simulink model "OMAP_ver_MIL10"  (R2018b)
settings: Solver=FixedStepDiscrete  StartTime=0.0  StopTime=10.0  FixedStep=0.01  RelTol=1e-3
undefined symbols (not defined in the file or in its folder): OMAP_Switch_EMS, OMAP_Switch_EPS, OMAP_Switch_ESC, OMAP_Switch_IC, OMAP_Switch_OTHER, TH_HMIClb_tiDgrdIconWarnHiDurT_C, TH_HMIClb_tiDgrdIconWarnLoDurT_C, TH_HMIClb_tiDgrdVocWarnDurT_C, TH_HMIClb_tiHndOffTxtWarnT_C, TH_HMIClb_tiHndOffVocWarnT_C, TH_HMIClb_tiSWALimFlgDetT_C, TH_HMIClb_tiTxtLimT_C
libraries: simulink x118
(part 2 of 9)

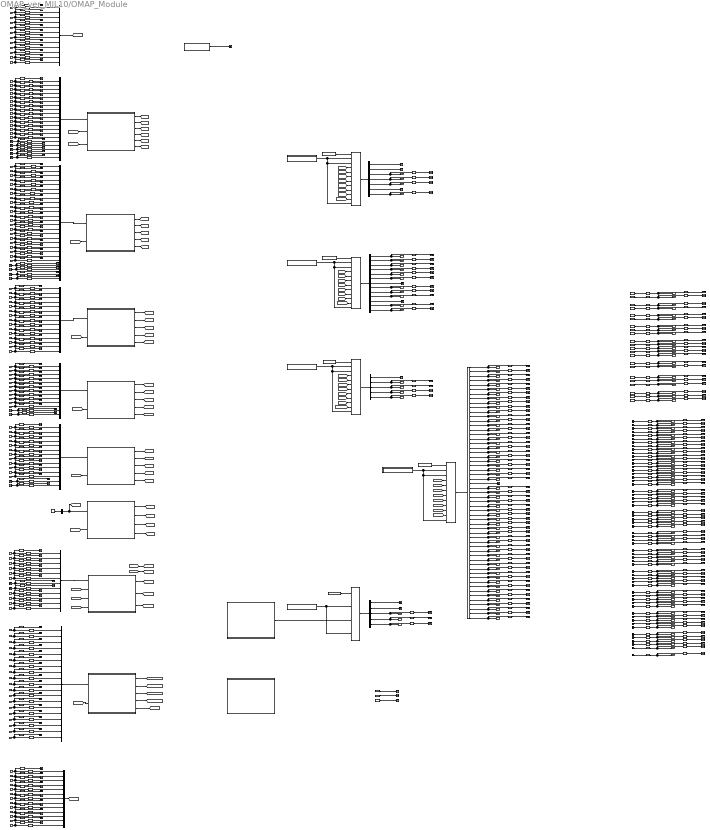
== system OMAP_ver_MIL10/OMAP_Module ==
  note: 仲裁#19——EW单功能调试模式
      | EMS、ESC、EPS、IC：只体现本功能的信号、且其他信号内容强制为“不动作”
  note: 仲裁#12——ACC单功能调试模式
      | EMS、ESC、EPS、IC：只体现本功能的信号、且其他信号内容强制为“不动作”
  note: 仲裁#17——ESA单功能调试模式
      | EMS、ESC、EPS、IC：只体现本功能的信号、且其他信号内容强制为“不动作”
  note: 仲裁#13——AEB单功能调试模式
      | EMS、ESC、EPS、IC：只体现本功能的信号、且其他信号内容强制为“不动作”
  note: 上面这是版本号
      | 蓝色的子系统是输入，橙色是仲裁输出，
      | 翠绿色的模块是标定量
  note: 仲裁#18——ICA单功能调试模式
      | EMS、ESC：只体现ACC的信号、且其他信号内容强制为“不动作”
      | EPS：只体现本功能的信号、且其他信号内容强制为“不动作”
      | IC：只体现本功能及ACC综合后的的信号、且其他信号内容强制为“不动作”
  note: 仲裁#16——ELK单功能调试模式
      | EMS、ESC、EPS、IC：只体现本功能的信号、且其他信号内容强制为“不动作”
  note: 仲裁#15——LKA单功能调试模式
      | EMS、ESC、EPS、IC：只体现本功能的信号、且其他信号内容强制为“不动作”
  note: 仲裁#14——JA单功能调试模式——
      | EMS、ESC、EPS、IC：只体现本功能的信号、且其他信号内容强制为“不动作”
  FDMMve_d_JaFcnConf : Inport  OutDataTypeStr=uint16
  FDMMve_d_AebFcnConf : Inport  Port=2  OutDataTypeStr=uint16
  FDMMve_d_EsaFcnConf : Inport  Port=3  OutDataTypeStr=uint16
  FDMMve_d_ElkFcnConf : Inport  Port=4  OutDataTypeStr=uint16
  FDMMve_d_LkaFcnConf : Inport  Port=5  OutDataTypeStr=uint16
  FDMMve_d_IcaFcnConf : Inport  Port=6  OutDataTypeStr=uint16
  FDMMve_d_AccFcnConf : Inport  Port=7  OutDataTypeStr=uint16
  FDMMve_d_LfFcnConf : Inport  Port=8  OutDataTypeStr=uint16
  FDMMve_d_AlcFcnConf : Inport  Port=9  OutDataTypeStr=uint16
  FDMMve_d_EwFcnConf : Inport  Port=10  OutDataTypeStr=uint16
  FDMMve_g_Adas2Fapa : Inport  Port=11  OutDataTypeStr=uint32
  FDMMve_d_SignalTStamp : Inport  Port=12  OutDataTypeStr=uint16
  ACCSve_d_ACC_State : Inport  Port=13  OutDataTypeStr=uint16
  ACCSve_g_ACC_TqReq : Inport  Port=14  OutDataTypeStr=single
  ACCSve_d_ACC_TqFlag : Inport  Port=15  OutDataTypeStr=uint16
  ACCSve_g_ACC_DecReq : Inport  Port=16  OutDataTypeStr=single
  ACCSve_d_ACC_DecFlag : Inport  Port=17  OutDataTypeStr=uint16
  ACCSve_d_CIPV_ID : Inport  Port=18  OutDataTypeStr=uint16
  ACCSve_d_ACCActive_Signal : Inport  Port=19  OutDataTypeStr=uint16
  ACCSve_d_ACC_go_request : Inport  Port=20  OutDataTypeStr=uint16
  ACCSve_d_VelocitySet : Inport  Port=21  OutDataTypeStr=uint16
  ACCSve_d_HeadWaySet : Inport  Port=22  OutDataTypeStr=uint16
  ACCSve_d_SignalTStamp : Inport  Port=23  OutDataTypeStr=uint16
  ACCSve_d_ACC_ICA_Flag : Inport  Port=24  OutDataTypeStr=uint16
  ACCSve_d_ACC_ESCDriveOff : Inport  Port=25  OutDataTypeStr=uint16
  ACCSve_d_ACC_ESCHoldReq : Inport  Port=26  OutDataTypeStr=uint16
  ACCSve_d_ACC_EPBReq : Inport  Port=27  OutDataTypeStr=uint16
  AEBSve_d_Prefill_request : Inport  Port=28  OutDataTypeStr=uint16
  AEBSve_d_functionFARCState : Inport  Port=29  OutDataTypeStr=uint16
  AEBSve_g_DecSetpoint : Inport  Port=30  OutDataTypeStr=single
  AEBSve_d_MDDdecRequest : Inport  Port=31  OutDataTypeStr=uint16
  AEBSve_d_MDDdecType : Inport  Port=32  OutDataTypeStr=uint16
  AEBSve_d_ESCDriveOff : Inport  Port=33  OutDataTypeStr=uint16
  AEBSve_d_ESCHoldReq : Inport  Port=34  OutDataTypeStr=uint16
  AEBSve_d_HapticAlarm : Inport  Port=35  OutDataTypeStr=uint16
  AEBSve_d_Braking_progress : Inport  Port=36  OutDataTypeStr=uint16
  AEBSve_d_AEBStatus : Inport  Port=37  OutDataTypeStr=uint16
  AEBSve_d_FCWStatus : Inport  Port=38  OutDataTypeStr=uint16
  AEBSve_d_AEBSwitchStatus : Inport  Port=39  OutDataTypeStr=uint16
  AEBSve_d_AEBFaultStatus : Inport  Port=40  OutDataTypeStr=uint16
  AEBSve_d_AEBAlertReq : Inport  Port=41  OutDataTypeStr=uint16
  AEBSve_d_AEBTips : Inport  Port=42  OutDataTypeStr=uint16
  AEBSve_d_SignalTStamp : Inport  Port=43  OutDataTypeStr=uint16
  AEBSve_d_JABS_AlertSign : Inport  Port=44  OutDataTypeStr=uint16
  AEBSve_d_JABS_SwitchStatus : Inport  Port=45  OutDataTypeStr=uint16
  AEBSve_d_JABS_FltStatus : Inport  Port=46  OutDataTypeStr=uint16
  AEBSve_d_JABS_AlertReq : Inport  Port=47  OutDataTypeStr=uint16
  AEBSve_d_JABS_HapticAlarm : Inport  Port=48  OutDataTypeStr=uint16
  AEBSve_d_JABS_Tips : Inport  Port=49  OutDataTypeStr=uint16
  JABSve_d_DbPrefillReq : Inport  Port=50  OutDataTypeStr=uint16
  JABSve_d_DbFunFARCSta : Inport  Port=51  OutDataTypeStr=uint16
  JABSve_g_DbDecSetpoint : Inport  Port=52  OutDataTypeStr=single
  JABSve_d_DbMDDdecRequest : Inport  Port=53  OutDataTypeStr=uint16
  JABSve_d_DbMDDdecType : Inport  Port=54  OutDataTypeStr=uint16
  JABSve_d_DbHapticAlarm : Inport  Port=55  OutDataTypeStr=uint16
  JABSve_d_DbBraking_progress : Inport  Port=56  OutDataTypeStr=uint16
  JABSve_d_DbSignalTStamp : Inport  Port=57  OutDataTypeStr=uint16
  JABSve_d_DbJACWStatus : Inport  Port=58  OutDataTypeStr=uint16
  JABSve_d_DbSwitchStatus : Inport  Port=59  OutDataTypeStr=uint16
  JABSve_d_DbFltStatus : Inport  Port=60  OutDataTypeStr=uint16
  JABSve_d_DbAlertReq : Inport  Port=61  OutDataTypeStr=uint16
  JABSve_d_DbTips : Inport  Port=62  OutDataTypeStr=uint16
  JABSve_d_DbESCDriveOff : Inport  Port=63  OutDataTypeStr=uint16
  JABSve_d_DbESCHoldReq : Inport  Port=64  OutDataTypeStr=uint16
  LKASve_y_Vehicle_Lane_Display : Inport  Port=65  OutDataTypeStr=uint8
  LKASve_y_LDW_Status_Display : Inport  Port=66  OutDataTypeStr=uint8
  LKASve_y_LKA_Status_Display : Inport  Port=67  OutDataTypeStr=uint8
  LKASve_y_LDW_Flag : Inport  Port=68  OutDataTypeStr=uint8
  LKASve_y_Hands_Off_Warning : Inport  Port=69  OutDataTypeStr=uint8
  LKASve_y_LKA_Action_Indication : Inport  Port=70  OutDataTypeStr=uint8
  LKASve_y_HMI_Popup_Status : Inport  Port=71  OutDataTypeStr=uint8
  LKASve_y_EPS_State_Control : Inport  Port=72  OutDataTypeStr=uint8
  LKASve_g_LKA_SWA_Control : Inport  Port=73  OutDataTypeStr=single
  LKASve_g_EPS_Factor_Control : Inport  Port=74  OutDataTypeStr=single
  LKASve_y_EPS_LKA_Control : Inport  Port=75  OutDataTypeStr=uint8
  ELKSve_y_state_ELK_function : Inport  Port=76  OutDataTypeStr=uint8
  ELKSve_y_ELK_HapticAlarmReq : Inport  Port=77  OutDataTypeStr=uint8
  ELKSve_y_Hands_Off_Warning : Inport  Port=78  OutDataTypeStr=uint8
  ELKSve_y_ELK_Action_Indication : Inport  Port=79  OutDataTypeStr=uint8
  ELKSve_y_HMI_Popup_Status : Inport  Port=80  OutDataTypeStr=uint8
  ELKSve_y_EPS_State_Control : Inport  Port=81  OutDataTypeStr=uint8
  ELKSve_g_ELK_SWA_Control : Inport  Port=82  OutDataTypeStr=single
  ELKSve_g_EPS_Factor_Control : Inport  Port=83  OutDataTypeStr=single
  ELKSve_y_EPS_ELK_Control : Inport  Port=84  OutDataTypeStr=uint8
  ELKSve_y_ELK_VehicleLaneDisp : Inport  Port=85  OutDataTypeStr=uint8
  ELKSve_y_ELK_ELKSts : Inport  Port=86  OutDataTypeStr=uint8
  ELKSve_y_SignalTStamp : Inport  Port=87  OutDataTypeStr=uint8
  ICABva_d_PathQI : Inport  Port=88  OutDataTypeStr=uint16
  ICABve_d_SignalTStamp : Inport  Port=89  OutDataTypeStr=uint16
  ICABva_d_ICAB2HMI : Inport  Port=90  OutDataTypeStr=uint16
  ICABve_g_SteerAngleCmd : Inport  Port=91  OutDataTypeStr=single
  ICABve_d_ICAMode : Inport  Port=92  OutDataTypeStr=uint16
  ICABve_d_ICAState : Inport  Port=93  OutDataTypeStr=uint16
  ICADva_d_DecionState : Inport  Port=94  OutDataTypeStr=uint16
  ICADva_d_DecionCMD : Inport  Port=95  OutDataTypeStr=uint16
  ICADva_d_LCRecommend : Inport  Port=96  OutDataTypeStr=uint16
  ICADve_d_SignalTStamp : Inport  Port=97  OutDataTypeStr=uint16
  EWWWve_y_LCW_M_SystemWorkingSt : Inport  Port=98  OutDataTypeStr=uint8
  EWWWve_y_RCTA_M_SystemWorkingSt : Inport  Port=99  OutDataTypeStr=uint8
  EWWWve_y_DOW_M_SystemWorkingSt : Inport  Port=100  OutDataTypeStr=uint8
  EWWWve_y_BSD_M_ErrorSt : Inport  Port=101  OutDataTypeStr=uint8
  EWWWve_y_BSD_M_LCAWarning : Inport  Port=102  OutDataTypeStr=uint8
  EWWWve_y_BSD_M_DoorOpenWarning : Inport  Port=103  OutDataTypeStr=uint8
  EWWWve_y_BSD_M_RCTAWarning : Inport  Port=104  OutDataTypeStr=uint8
  EWWWve_y_BSD_S_LCAWarning : Inport  Port=105  OutDataTypeStr=uint8
  EWWWve_y_BSD_S_DoorOpenWarning : Inport  Port=106  OutDataTypeStr=uint8
  EWWWve_y_BSD_S_RCTAWarning : Inport  Port=107  OutDataTypeStr=uint8
  EWWWve_y_SRR_LF_FCTAWorkingSt : Inport  Port=108  OutDataTypeStr=uint8
  EWWWve_y_SRR_LF_ErrorSt : Inport  Port=109  OutDataTypeStr=uint8
  EWWWve_y_SRR_LF_FCTAWarning : Inport  Port=110  OutDataTypeStr=uint8
  EWWWve_y_SRR_RF_FCTAWarning : Inport  Port=111  OutDataTypeStr=uint8
  EWWWve_y_SRR_SystemState : Inport  Port=112  OutDataTypeStr=uint8
  EWWWve_y_BSD_S_SystemStateInfo : Inport  Port=113  OutDataTypeStr=uint8
  EWWWve_y_BSD_SystemStateInfo : Inport  Port=114  OutDataTypeStr=uint8
  EWWWve_y_SRR_LF_SystemStateInfo : Inport  Port=115  OutDataTypeStr=uint8
  EWWWve_y_SRR_RF_SystemStateInfo : Inport  Port=116  OutDataTypeStr=uint8
  IMAPve_d_EPS_LKA_State : Inport  Port=117  OutDataTypeStr=uint16
  IMAPve_g_ESC_LonAcc : Inport  Port=118  OutDataTypeStr=single
  IMAPva_d_obj_id : Inport  Port=119  OutDataTypeStr=uint16
  IMAPva_g_obj_pos_x : Inport  Port=120  OutDataTypeStr=single
  IMAPve_d_ESC_Veh_Standstill : Inport  Port=121  OutDataTypeStr=uint16
  IMAPve_g_L0_C0 : Inport  Port=122  OutDataTypeStr=single
  IMAPve_g_L0_C1 : Inport  Port=123  OutDataTypeStr=single
  IMAPve_g_L0_C2 : Inport  Port=124  OutDataTypeStr=single
  IMAPve_g_L0_C3 : Inport  Port=125  OutDataTypeStr=single
  IMAPve_g_R0_C0 : Inport  Port=126  OutDataTypeStr=single
  IMAPve_g_R0_C1 : Inport  Port=127  OutDataTypeStr=single
  IMAPve_g_R0_C2 : Inport  Port=128  OutDataTypeStr=single
  IMAPve_g_R0_C3 : Inport  Port=129  OutDataTypeStr=single
  ACCS_Direct : Subsystem
  AEBS_Direct : Subsystem
  Bus Creator : BusCreator  Inputs=1
  Bus Selector : BusSelector  OutputSignals=OMAPve_y_ACC_Engine_Start_Request_1,OMAPve_g_PotACCTqReq_1,OMAPve_g_ACCTqReq_1,OMAPve_y_Powertrain_torquewheel_request_1,OMAPve_g_TminUp_or_downGear_1,OMAPve_y_stAcvTqWhlPTPotReq_1,OMAPve_y_Function_Acc_status_1
  Bus Selector1 : BusSelector  OutputSignals=OMAPve_g_Deceleration_setpoint_device_1,OMAPve_y_MDD_Decelerationcontrol_request_1,OMAPve_y_Prefill_request_1,OMAPve_y_ADAS_ESCDriveOff,OMAPve_y_ADAS_ESCHoldReq,OMAPve_y_MDD_deceleration_type_1,OMAPve_y_State_of_the_functionFARC_det_1,OMAPve_y_AEB_Status_1,OMAPve_y_Decel_Request_1,OMAPve_y_AEB_Braking_progress_1,OMAPve_y_FCW_Status_1,OMAPve_y_Haptic_Alarm_1,OMAPve_y_ADAS_ACCRequestEPB
  Bus Selector2 : BusSelector  OutputSignals=OMAPve_y_Power_steering_power_cut3F2_2,OMAPve_y_General_state_of_LKA_function3F2_2,OMAPve_g_Coefficient_toregulate_EPS_2,OMAPve_g_Column_angle_setpoint3F2_2,OMAPve_y_Permit_to_know_if_LKA_or_LPA3F2_2
  Bus Selector3 : BusSelector  OutputSignals=OMAPve_y_TSR_Vision_Only_Sign_Type_2,OMAPve_y_ISA_Popup_text_2,OMAPve_y_ISA_Sign_Type_2,OMAPve_y_ISA_Status_2,OMAPve_y_ISA_Value_2,OMAPve_y_ACC_DesiredHeadway_Display_2,OMAPve_y_ACC_DesiredHeadway_Icon_Basic_2,OMAPve_y_ACC_Desired_Set_Speed_2,OMAPve_y_ACC_Set_Speed_Display_2,OMAPve_y_ACC_Vehicle_Icon_Display_2,OMAPve_y_RVVACC_Vehiclespeed_request_type_2,OMAPve_y_ACC_Pop_Up_Message_2,OMAPve_y_AEB_Alert_Req_2,OMAPve_y_AEB_Fault_Status_2,OMAPve_y_AEB_Switch_Status_2,OMAPve_y_AEB_tips_2,OMAPve_y_ACC_HMI_TgtDisp_Flag_2,OMAPve_y_TARGET_POSITION_2,OMAPve_y_Hands_off_warning_2,OMAPve_y_HMI_Popup_Status_2,OMAPve_y_Vehicle_Lane_Display_2,OMAPve_y_LDW_Flag_2,OMAPve_y_LDW_Status_Display_2,OMAPve_y_LKA_Mode_from_Camera_2,OMAPve_y_LKA_Status_Display_2,OMAPve_y_LKA_Switch_State_2,OMAPve_y_LKA_action_indication_2,OMAPve_y_ADAS_ELKSts_2,OMAPve_y_ICA_HMI_Txt_Disp_2,OMAPve_y_TJA_status_icon_2,OMAPve_y_ADAS_SRR_SystemState,OMAPve_y_ADAS_LeftLEDWarningSt,OMAPve_y_ADAS_RighrLEDWarningSt,OMAPve_y_ADAS_BSD_SystemStInfo,OMAPve_y_ADAS_BSD_LCWWorkingSt,OMAPve_y_ADAS_BSD_ErrorSt,OMAPve_y_ADAS_BSD_LCAWarning,OMAPve_y_ADAS_BSD_DoorOpenWrn,OMAPve_y_ADAS_BSD_RCTAWarning,OMAPve_y_ADAS_BSD_DOWWorkingSt,OMAPve_y_ADAS_BSD_RCTAWorkingSt,OMAPve_y_ADAS_BSD_S_SystStInfo,OMAPve_y_ADAS_BSD_S_LCWWorkSt,OMAPve_y_ADAS_BSD_S_ErrorSt,OMAPve_y_ADAS_BSD_S_LCAWarning,OMAPve_y_ADAS_BSD_S_DoorOpenWrn,OMAPve_y_ADAS_BSD_S_RCTAWarning,OMAPve_y_ADAS_BSD_S_DOWWorkSt,OMAPve_y_ADAS_BSD_S_RCTAWorkSt,OMAPve_y_ADAS_SRR_LF_SystStInfo,OMAPve_y_ADAS_SRR_LF_SystWorkSt,OMAPve_y_ADAS_SRR-LF_ErrorSt,OMAPve_y_ADAS_SRR_LF_FCTAWrn,OMAPve_y_ADAS_SRR_RF_SystStInfo,OMAPve_y_ADAS_SRR_RF_SystWorkSt,OMAPve_y_ADAS_SRR-RF_ErrorSt,OMAPve_y_ADAS_SRR_RF_FCTAWrn
  Bus Selector4 : BusSelector  OutputSignals=OMAPve_y_ABS_ESP_power_cut_request2_2,OMAPve_y_ASR_connection_dis_demand2_2,OMAPve_y_TYPE_RAPPORT_2,OMAPve_y_ECU_operating_phase_2,OMAPve_y_Radar_State_2
  Bus_ACCS : BusCreator  Inputs=20
  Bus_AEBS : BusCreator  Inputs=26
  Bus_ELKS : BusCreator  Inputs=14
  Bus_EW : BusCreator  Inputs=19
  Bus_FDMM : BusCreator  Inputs=12
  Bus_ICA : BusCreator  Inputs=12
  Bus_IMAP : BusCreator  Inputs=13
  Bus_JABS : BusCreator  Inputs=15
  Bus_LKAS : BusCreator  Inputs=13
  CHecksum_Rollingcounter : Subsystem
  Constant : Constant  Value=OMAP_Switch_EMS  OutDataTypeStr=uint8
  Constant1 : Constant  Value=OMAP_Switch_ESC  OutDataTypeStr=uint8
  Constant2 : Constant  Value=OMAP_Switch_EPS  OutDataTypeStr=uint8
  Constant3 : Constant  Value=OMAP_Switch_IC  OutDataTypeStr=uint8
  Constant4 : Constant  Value=OMAP_Switch_OTHER  OutDataTypeStr=uint8
  Constant5 : Constant  OutDataTypeStr=uint8
  Constant6 : Constant  Value=920  OutDataTypeStr=uint16
  Data Type Conversion{,1..10,13..21,23..31,55,57..58,60,62..63,78..86,89..91,93,95..98,100,149..160,162..165,167..177,180} (81 alike) : DataTypeConversion  OutDataTypeStr=uint16
  Data Type Conversion{54,56,88,92,94,99,101..110,144..145,161,166,179,182} (22 alike) : DataTypeConversion  OutDataTypeStr=single
  Data Type Conversion{11..12,87,111..143,146..148,178} (40 alike) : DataTypeConversion  OutDataTypeStr=uint8
  Data Type Conversion22 : DataTypeConversion  OutDataTypeStr=uint32
  Default_EMS : Subsystem
  Default_EPS : Subsystem
  Default_ESC : Subsystem
  Default_IC : Subsystem
  Default_OTHER : Subsystem
  ELKS_Direct : Subsystem
  ESAS_Direct : Subsystem
  EW_ISA_TSR_Direct : Subsystem
  Ground{,1..14} (15 alike) : Ground
  ICA_Direct_G59 : Subsystem
  Index Vector{,1..3} (4 alike) : MultiPortSwitch  DataPortOrder=Zero-based contiguous  Inputs=11  zeroidx=on
  Index Vector4 : MultiPortSwitch  DataPortOrder=Zero-based contiguous  zeroidx=on
  JABS_Direct : Subsystem
  LKAS_Direct : Subsystem
  OMAPve_g_ADAS_ESATorqueReq1 : Constant  Value=0  OutDataTypeStr=single
  OMAPve_g_ADAS_L0_C0_COEF_2 : Ground
  OMAPve_g_ADAS_L0_C1_COEF_2 : Ground
  OMAPve_g_ADAS_L0_C2_COEF_2 : Ground
  OMAPve_g_ADAS_L0_C3_COEF_2 : Ground
  OMAPve_g_ADAS_OBJ01_LatDis_2 : Ground
  OMAPve_g_ADAS_OBJ01_LgtDis_2 : Ground
  OMAPve_g_ADAS_OBJ02_LatDis_2 : Ground
  OMAPve_g_ADAS_OBJ02_LgtDis_2 : Ground
  OMAPve_g_ADAS_OBJ03_LatDis_2 : Ground
  OMAPve_g_ADAS_OBJ03_LgtDis_2 : Ground
  OMAPve_g_ADAS_OBJ04_LatDis_2 : Ground
  OMAPve_g_ADAS_OBJ04_LgtDis_2 : Ground
  OMAPve_g_ADAS_OBJ05_LatDis_2 : Ground
  OMAPve_g_ADAS_OBJ05_LgtDis_2 : Ground
  OMAPve_g_ADAS_OBJ06_LatDis_2 : Ground
  OMAPve_g_ADAS_OBJ06_LgtDis_2 : Ground
  OMAPve_g_ADAS_R0_C0_COEF_2 : Ground
  OMAPve_g_ADAS_R0_C1_COEF_2 : Ground
  OMAPve_g_ADAS_R0_C2_COEF_2 : Ground
  OMAPve_g_ADAS_R0_C3_COEF_2 : Ground
  OMAPve_y_ADAS_ACCLateralDist1 : Constant  Value=0  OutDataTypeStr=int8
  OMAPve_y_ADAS_ACCLongiDist1 : Constant  Value=0  OutDataTypeStr=uint8
  OMAPve_y_ADAS_BackObjectLeft_2 : Ground
  OMAPve_y_ADAS_BackObjectRight_2 : Ground
  OMAPve_y_ADAS_ESAFaultSt1 : Constant  Value=0  OutDataTypeStr=uint8
  OMAPve_y_ADAS_ESARequest1 : Constant  Value=0  OutDataTypeStr=uint8
  OMAPve_y_ADAS_ESAState1 : Constant  Value=0  OutDataTypeStr=uint8
  OMAPve_y_ADAS_EngStartReqForSTT1 : Constant  Value=0  OutDataTypeStr=uint8
  OMAPve_y_ADAS_EngStopPmtForSTT1 : Constant  Value=0  OutDataTypeStr=uint8
  OMAPve_y_ADAS_FrontObj01Class_2 : Ground
  OMAPve_y_ADAS_FrontObj02Class_2 : Ground
  OMAPve_y_ADAS_FrontObj03Class_2 : Ground
  OMAPve_y_ADAS_FrontObj04Class_2 : Ground
  OMAPve_y_ADAS_FrontObj05Class_2 : Ground
  OMAPve_y_ADAS_FrontObj06Class_2 : Ground
  OMAPve_y_ADAS_FrontObject01Zone_2 : Ground
  OMAPve_y_ADAS_FrontObject02Zone_2 : Ground
  OMAPve_y_ADAS_FrontObject03Zone_2 : Ground
  OMAPve_y_ADAS_FrontObject04Zone_2 : Ground
  OMAPve_y_ADAS_FrontObject05Zone_2 : Ground
  OMAPve_y_ADAS_FrontObject06Zone_2 : Ground
  OMAPve_y_ADAS_HWAActionSts1 : Constant  Value=0  OutDataTypeStr=uint8
  OMAPve_y_ADAS_HWAMode1 : Constant  Value=0  OutDataTypeStr=uint8
  OMAPve_y_ADAS_HWATurnOnIdctr1 : Constant  Value=0  OutDataTypeStr=uint8
  OMAPve_y_ADAS_IHBC_Fuction_St1 : Constant  Value=0  OutDataTypeStr=uint8
  OMAPve_y_ADAS_IHBC_HB_Req1 : Constant  Value=0  OutDataTypeStr=uint8
  OMAPve_y_ADAS_ISLCDriverRemind1 : Constant  Value=0  OutDataTypeStr=uint8
  OMAPve_y_ADAS_ISLCState1 : Constant  Value=0  OutDataTypeStr=uint8
  OMAPve_y_ADAS_JAFaultSt1 : Constant  Value=0  OutDataTypeStr=uint8
  OMAPve_y_ADAS_L0LineType_2 : Ground
  OMAPve_y_ADAS_L0_LINE_TYPE_2 : Ground
  OMAPve_y_ADAS_L1LineType_2 : Ground
  OMAPve_y_ADAS_LCAPopupMessage1 : Constant  Value=0  OutDataTypeStr=uint8
  OMAPve_y_ADAS_LCAStatusDisplay1 : Constant  Value=0  OutDataTypeStr=uint8
  OMAPve_y_ADAS_LetfLigthControl1 : Constant  Value=0  OutDataTypeStr=uint8
  OMAPve_y_ADAS_LightControlValid1 : Constant  Value=0  OutDataTypeStr=uint8
  OMAPve_y_ADAS_LineCurveType_2 : Ground
  OMAPve_y_ADAS_OBJ01_Class_2 : Ground
  OMAPve_y_ADAS_OBJ01_ID_2 : Ground
  OMAPve_y_ADAS_OBJ01_Lane_2 : Ground
  OMAPve_y_ADAS_OBJ02_Class_2 : Ground
  OMAPve_y_ADAS_OBJ02_ID_2 : Ground
  OMAPve_y_ADAS_OBJ02_Lane_2 : Ground
  OMAPve_y_ADAS_OBJ03_Class_2 : Ground
  OMAPve_y_ADAS_OBJ03_ID_2 : Ground
  OMAPve_y_ADAS_OBJ03_Lane_2 : Ground
  OMAPve_y_ADAS_OBJ04_Class_2 : Ground
  OMAPve_y_ADAS_OBJ04_ID_2 : Ground
  OMAPve_y_ADAS_OBJ04_Lane_2 : Ground
  OMAPve_y_ADAS_OBJ05_Class_2 : Ground
  OMAPve_y_ADAS_OBJ05_ID_2 : Ground
  OMAPve_y_ADAS_OBJ05_Lane_2 : Ground
  OMAPve_y_ADAS_OBJ06_Class_2 : Ground
  OMAPve_y_ADAS_OBJ06_ID_2 : Ground
  OMAPve_y_ADAS_OBJ06_Lane_2 : Ground
  OMAPve_y_ADAS_R0LineType_2 : Ground
  OMAPve_y_ADAS_R0_LINE_TYPE_2 : Ground
  OMAPve_y_ADAS_R1LineType_2 : Ground
  OMAPve_y_ADAS_RightLigthControl1 : Constant  Value=0  OutDataTypeStr=uint8
  OMAPve_y_ADAS_State1 : Constant  Value=0  OutDataTypeStr=uint8
  OMAPve_y_Dead_man_dedicated_push_button2Num : Constant  Value=0  OutDataTypeStr=uint8
  OMAPve_y_EASYMOVE_powercut_request3F2Num : Constant  Value=0  OutDataTypeStr=uint8
  OMAPve_y_Trailer_Present3F2Num : Constant  Value=0  OutDataTypeStr=uint8
  OTHER_Default_Arbitration : Subsystem
  Terminator{,1..12} (13 alike) : Terminator
  ob_In_convert{1..10,12..13,15,17..29,31..51,53..64,88..90,92..97,117,119,121,130..138,143} (81 alike) : DataTypeConversion  OutDataTypeStr=uint16
  ob_In_convert{65..72,75..81,84..87,98..116,139,141} (40 alike) : DataTypeConversion  OutDataTypeStr=uint8
  ob_In_convert11 : DataTypeConversion  OutDataTypeStr=uint32
  ob_In_convert{14,16,30,52,73..74,82..83,91,118,120,122..129,140,142,144} (22 alike) : DataTypeConversion  OutDataTypeStr=single
  ob_In_terminator{1..144} (144 alike) : Terminator
  ob_convert{1..21,24,26..27,29..49,52..53,55..120,125,132..134,137..139,142..144,147..149,152..154,157..162,164..167,169..200,202,207,213..214,216,218..219,221,223..224,226,228..229,231,233..234,236,238..240} (191 alike) : DataTypeConversion  OutDataTypeStr=uint8
  ob_convert{23,25,28,50..51,54,121..124,126..131,135..136,140..141,145..146,150..151,155..156,168,201,203..206,208..212,215,217,220,222,225,227,230,232,235,237} (47 alike) : DataTypeConversion  OutDataTypeStr=single
  ob_convert163 : DataTypeConversion  OutDataTypeStr=int8
  ob_convert22 : DataTypeConversion  OutDataTypeStr=int8
  ob_terminator{1..159} (159 alike) : Terminator
  OMAPve_y_ADAS_TSRSignType : Outport
      settings: AttributesFormatString=%<Description>在G59上值的定义变更
  OMAPve_y_ADAS_ISAPopupMessage : Outport  Port=2
  OMAPve_y_ADAS_ISASignType : Outport  Port=3
  OMAPve_y_ADAS_ISAStatus : Outport  Port=4
  OMAPve_y_ADAS_ISAValue : Outport  Port=5
  OMAPve_y_ADAS_ISLCState : Outport  Port=6
  OMAPve_y_ADAS_ISLCDriverRemind : Outport  Port=7
  OMAPve_y_ADAS_ACCHeadwayDisplay : Outport  Port=8
  OMAPve_y_ADAS_ACCHeadwayIcon : Outport  Port=9
  OMAPve_y_ADAS_ACCSetSpeed : Outport  Port=10
  OMAPve_y_ADAS_ACCSetSpeedDis : Outport  Port=11
  OMAPve_y_ADAS_ACCStatusIconDis : Outport  Port=12
  OMAPve_y_ADAS_ACC_RVVReqType : Outport  Port=13
  OMAPve_y_ADAS_ACCMessagePrompt : Outport  Port=14
      settings: AttributesFormatString=%<Description>在G59值的定义变了
  OMAPve_y_ADAS_AEBAlertReq : Outport  Port=15
      settings: AttributesFormatString=%<Description>在G59新增了值3：JA报警
  OMAPve_y_ADAS_AEBFaultStatus : Outport  Port=16
  OMAPve_y_ADAS_AEBSwitchStatus : Outport  Port=17
  OMAPve_y_ADAS_AEBMassageDisp : Outport  Port=18
  OMAPve_y_ADAS_HMITargetDispFlag : Outport  Port=19
  OMAPve_y_ADAS_TargetPosition : Outport  Port=20
  OMAPve_y_ADAS_ACCLongiDist : Outport  Port=21
  OMAPve_y_ADAS_ACCLateralDist : Outport  Port=22
  OMAPve_g_ADAS_ACCTorqueReq : Outport  Port=23
  OMAPve_y_ADAS_TorqueActivReq : Outport  Port=24
  OMAPve_g_ADAS_DownorUpGearMinTime : Outport  Port=25
  OMAPve_y_ADAS_UpDownGearChange : Outport  Port=26
  OMAPve_y_ADAS_ACCState : Outport  Port=27
  OMAPve_g_ADAS_DecelerationSet : Outport  Port=28
  OMAPve_y_ADAS_DeclControlReq : Outport  Port=29
  OMAPve_y_ADAS_PrefillRequest : Outport  Port=30
  OMAPve_y_ADAS_ESCDriveOff : Outport  Port=31
  OMAPve_y_ADAS_ESCHoldReq : Outport  Port=32
  OMAPve_y_ADAS_DecelerationType : Outport  Port=33
  OMAPve_y_ADAS_AEBState : Outport  Port=34
      settings: AttributesFormatString=%<Description>在G59值的定义改变
  OMAPve_y_ADAS_BrakeRequest : Outport  Port=35
  OMAPve_y_ADAS_AEBBrakingProg : Outport  Port=36
  OMAPve_y_ADAS_HapticAlarmReq : Outport  Port=37
  OMAPve_y_ADAS_Handsoffwarning : Outport  Port=38
  OMAPve_y_ADAS_HMIPopupMassage : Outport  Port=39
  OMAPve_y_ADAS_VehicleLaneDisp : Outport  Port=40
      settings: AttributesFormatString=%<Description>在G59值的定义变了
  OMAPve_y_ADAS_LDWWarningSt : Outport  Port=41
  OMAPve_y_ADAS_LDWStatusDisplay : Outport  Port=42
  OMAPve_y_ADAS_LKAMode : Outport  Port=43
  OMAPve_y_ADAS_LKAStatusDisplay : Outport  Port=44
  OMAPve_y_ADAS_LKASwitchState : Outport  Port=45
  OMAPve_y_ADAS_ELKSts : Outport  Port=46
  OMAPve_y_ADAS_LCAStatusDisplay : Outport  Port=47
  OMAPve_y_ADAS_LCAPopupMessage : Outport  Port=48
  OMAPve_y_ADAS_LKAState : Outport  Port=49
      settings: AttributesFormatString=%<Description>在G59改了信号周期。内容没变
  OMAPve_g_ADAS_LKATorqFactReq : Outport  Port=50
      settings: AttributesFormatString=%<Description>在G59改了信号周期。内容没变
  OMAPve_g_ADAS_LKAAngleReq : Outport  Port=51
      settings: AttributesFormatString=%<Description>在G59改了信号周期。内容没变
  OMAPve_y_ADAS_LKAActivation : Outport  Port=52
  OMAPve_y_ADAS_ESAState : Outport  Port=53
  OMAPve_g_ADAS_ESATorqueReq : Outport  Port=54
  OMAPve_y_ADAS_ESARequest : Outport  Port=55
  OMAPve_y_ADAS_ICAMassageDisp : Outport  Port=56
      settings: AttributesFormatString=%<Description>在G59值的定义变了
  OMAPve_y_ADAS_ICAStatusIcon : Outport  Port=57
  OMAPve_y_ADAS_HWAMode : Outport  Port=58
  OMAPve_y_ADAS_HWATurnOnIdctr : Outport  Port=59
  OMAPve_y_ADAS_ESAFaultSt : Outport  Port=60
  OMAPve_y_ADAS_JAFaultSt : Outport  Port=61
  OMAPve_y_ADAS_HWAActionSts : Outport  Port=62
  OMAPve_y_ADAS_OperatingStatus : Outport  Port=63
  OMAPve_y_ADAS_IHBC_HB_Req : Outport  Port=64
  OMAPve_y_ADAS_IHBC_Fuction_St : Outport  Port=65
  OMAPve_y_ADAS_Radar_State : Outport  Port=66
  OMAPve_y_ADAS_ACCRequestEPB : Outport  Port=67
  OMAPve_y_ADAS_EngStartReqForSTT : Outport  Port=68
  OMAPve_y_ADAS_EngStopPmtForSTT : Outport  Port=69
  OMAPve_y_ADAS_State : Outport  Port=70
  OMAPve_y_ADAS_LetfLigthControl : Outport  Port=71
  OMAPve_y_ADAS_RightLigthControl : Outport  Port=72
  OMAPve_y_ADAS_LightControlValid : Outport  Port=73
  OMAPve_y_ADAS_SRR_SystemState : Outport  Port=74
  OMAPve_y_ADAS_LeftLEDWarningSt : Outport  Port=75
  OMAPve_y_ADAS_RighrLEDWarningSt : Outport  Port=76
  OMAPve_y_ADAS_BSD_SystemStInfo : Outport  Port=77
  OMAPve_y_ADAS_BSD_LCWWorkingSt : Outport  Port=78
  OMAPve_y_ADAS_BSD_ErrorSt : Outport  Port=79
  OMAPve_y_ADAS_BSD_LCAWarning : Outport  Port=80
  OMAPve_y_ADAS_BSD_DoorOpenWrn : Outport  Port=81
  OMAPve_y_ADAS_BSD_RCTAWarning : Outport  Port=82
  OMAPve_y_ADAS_BSD_DOWWorkingSt : Outport  Port=83
  OMAPve_y_ADAS_BSD_RCTAWorkingSt : Outport  Port=84
  OMAPve_y_ADAS_BSD_S_SystStInfo : Outport  Port=85
  OMAPve_y_ADAS_BSD_S_LCWWorkSt : Outport  Port=86
  OMAPve_y_ADAS_BSD_S_ErrorSt : Outport  Port=87
  OMAPve_y_ADAS_BSD_S_LCAWarning : Outport  Port=88
  OMAPve_y_ADAS_BSD_S_DoorOpenWrn : Outport  Port=89
  OMAPve_y_ADAS_BSD_S_RCTAWarning : Outport  Port=90
  OMAPve_y_ADAS_BSD_S_DOWWorkSt : Outport  Port=91
  OMAPve_y_ADAS_BSD_S_RCTAWorkSt : Outport  Port=92
  OMAPve_y_ADAS_SRR_LF_SystStInfo : Outport  Port=93
  OMAPve_y_ADAS_SRR_LF_SystWorkSt : Outport  Port=94
  OMAPve_y_ADAS_SRR_LF_ErrorSt : Outport  Port=95
  OMAPve_y_ADAS_SRR_LF_FCTAWrn : Outport  Port=96
  OMAPve_y_ADAS_SRR_RF_SystStInfo : Outport  Port=97
  OMAPve_y_ADAS_SRR_RF_SystWorkSt : Outport  Port=98
  OMAPve_y_ADAS_SRR_RF_ErrorSt : Outport  Port=99
  OMAPve_y_ADAS_SRR_RF_FCTAWrn : Outport  Port=100
  OMAPve_y_ADAS_L0LineType : Outport  Port=101
  OMAPve_y_ADAS_L1LineType : Outport  Port=102
  OMAPve_y_ADAS_R0LineType : Outport  Port=103
  OMAPve_y_ADAS_R1LineType : Outport  Port=104
  OMAPve_y_ADAS_LineCurveType : Outport  Port=105
  OMAPve_y_ADAS_FrontObject01Zone : Outport  Port=106
  OMAPve_y_ADAS_FrontObj01Class : Outport  Port=107
  OMAPve_y_ADAS_FrontObject02Zone : Outport  Port=108
  OMAPve_y_ADAS_FrontObj02Class : Outport  Port=109
  OMAPve_y_ADAS_FrontObject03Zone : Outport  Port=110
  OMAPve_y_ADAS_FrontObj03Class : Outport  Port=111
  OMAPve_y_ADAS_FrontObject04Zone : Outport  Port=112
  OMAPve_y_ADAS_FrontObj04Class : Outport  Port=113
  OMAPve_y_ADAS_FrontObject05Zone : Outport  Port=114
  OMAPve_y_ADAS_FrontObj05Class : Outport  Port=115
  OMAPve_y_ADAS_FrontObject06Zone : Outport  Port=116
  OMAPve_y_ADAS_FrontObj06Class : Outport  Port=117
  OMAPve_y_ADAS_BackObjectLeft : Outport  Port=118
  OMAPve_y_ADAS_BackObjectRight : Outport  Port=119
  OMAPve_y_ADAS_L0_LINE_TYPE : Outport  Port=120
  OMAPve_g_ADAS_L0_C0_COEF : Outport  Port=121
  OMAPve_g_ADAS_L0_C1_COEF : Outport  Port=122
  OMAPve_g_ADAS_L0_C2_COEF : Outport  Port=123
  OMAPve_g_ADAS_L0_C3_COEF : Outport  Port=124
  OMAPve_y_ADAS_R0_LINE_TYPE : Outport  Port=125
  OMAPve_g_ADAS_R0_C0_COEF : Outport  Port=126
  OMAPve_g_ADAS_R0_C1_COEF : Outport  Port=127
  OMAPve_g_ADAS_R0_C2_COEF : Outport  Port=128
  OMAPve_g_ADAS_R0_C3_COEF : Outport  Port=129
  OMAPve_g_ADAS_OBJ01_LatDis : Outport  Port=130
  OMAPve_g_ADAS_OBJ01_LgtDis : Outport  Port=131
  OMAPve_y_ADAS_OBJ01_Class : Outport  Port=132
  OMAPve_y_ADAS_OBJ01_ID : Outport  Port=133
  OMAPve_y_ADAS_OBJ01_Lane : Outport  Port=134
  OMAPve_g_ADAS_OBJ02_LatDis : Outport  Port=135
  OMAPve_g_ADAS_OBJ02_LgtDis : Outport  Port=136
  OMAPve_y_ADAS_OBJ02_Class : Outport  Port=137
  OMAPve_y_ADAS_OBJ02_ID : Outport  Port=138
  OMAPve_y_ADAS_OBJ02_Lane : Outport  Port=139
  OMAPve_g_ADAS_OBJ03_LatDis : Outport  Port=140
  OMAPve_g_ADAS_OBJ03_LgtDis : Outport  Port=141
  OMAPve_y_ADAS_OBJ03_Class : Outport  Port=142
  OMAPve_y_ADAS_OBJ03_ID : Outport  Port=143
  OMAPve_y_ADAS_OBJ03_Lane : Outport  Port=144
  OMAPve_g_ADAS_OBJ04_LatDis : Outport  Port=145
  OMAPve_g_ADAS_OBJ04_LgtDis : Outport  Port=146
  OMAPve_y_ADAS_OBJ04_Class : Outport  Port=147
  OMAPve_y_ADAS_OBJ04_ID : Outport  Port=148
  OMAPve_y_ADAS_OBJ04_Lane : Outport  Port=149
  OMAPve_g_ADAS_OBJ05_LatDis : Outport  Port=150
  OMAPve_g_ADAS_OBJ05_LgtDis : Outport  Port=151
  OMAPve_y_ADAS_OBJ05_Class : Outport  Port=152
  OMAPve_y_ADAS_OBJ05_ID : Outport  Port=153
  OMAPve_y_ADAS_OBJ05_Lane : Outport  Port=154
  OMAPve_g_ADAS_OBJ06_LatDis : Outport  Port=155
  OMAPve_g_ADAS_OBJ06_LgtDis : Outport  Port=156
  OMAPve_y_ADAS_OBJ06_Class : Outport  Port=157
  OMAPve_y_ADAS_OBJ06_ID : Outport  Port=158
  OMAPve_y_ADAS_OBJ06_Lane : Outport  Port=159
  wires:
  OMAPve_y_ADAS_ISLCState1/1 -> ob_convert160/1
  OMAPve_y_ADAS_ISLCDriverRemind1/1 -> ob_convert161/1
  OMAPve_y_ADAS_ACCLongiDist1/1 -> ob_convert162/1
  OMAPve_y_ADAS_ACCLateralDist1/1 -> ob_convert163/1
  OMAPve_y_ADAS_LCAStatusDisplay1/1 -> ob_convert164/1
  OMAPve_y_ADAS_LCAPopupMessage1/1 -> ob_convert165/1
  OMAPve_y_ADAS_ESAState1/1 -> ob_convert166/1
  OMAPve_g_ADAS_ESATorqueReq1/1 -> ob_convert168/1
  OMAPve_y_ADAS_ESARequest1/1 -> ob_convert167/1
  OMAPve_y_ADAS_HWAMode1/1 -> ob_convert169/1
  OMAPve_y_ADAS_HWATurnOnIdctr1/1 -> ob_convert170/1
  OMAPve_y_ADAS_ESAFaultSt1/1 -> ob_convert171/1
  OMAPve_y_ADAS_JAFaultSt1/1 -> ob_convert172/1
  OMAPve_y_ADAS_HWAActionSts1/1 -> ob_convert173/1
  OMAPve_y_ADAS_IHBC_HB_Req1/1 -> ob_convert174/1
  OMAPve_y_ADAS_IHBC_Fuction_St1/1 -> ob_convert175/1
  OMAPve_y_ADAS_EngStartReqForSTT1/1 -> ob_convert176/1
  OMAPve_y_ADAS_EngStopPmtForSTT1/1 -> ob_convert177/1
  OMAPve_y_ADAS_State1/1 -> ob_convert178/1
  OMAPve_y_ADAS_LetfLigthControl1/1 -> ob_convert179/1
  OMAPve_y_ADAS_RightLigthControl1/1 -> ob_convert180/1
  OMAPve_y_ADAS_LightControlValid1/1 -> ob_convert181/1
  Bus Selector3/34 -> OMAPve_y_ADAS_BSD_SystemStInfo/1, ob_convert77/1  "<OMAPve_y_ADAS_BSD_SystemStInfo>"
  Bus Selector3/35 -> OMAPve_y_ADAS_BSD_LCWWorkingSt/1, ob_convert78/1  "<OMAPve_y_ADAS_BSD_LCWWorkingSt>"
  Bus Selector3/46 -> OMAPve_y_ADAS_BSD_S_DoorOpenWrn/1, ob_convert89/1  "<OMAPve_y_ADAS_BSD_S_DoorOpenWrn>"
  Bus Selector3/50 -> OMAPve_y_ADAS_SRR_LF_SystStInfo/1, ob_convert93/1  "<OMAPve_y_ADAS_SRR_LF_SystStInfo>"
  Bus Selector3/51 -> OMAPve_y_ADAS_SRR_LF_SystWorkSt/1, ob_convert94/1  "<OMAPve_y_ADAS_SRR_LF_SystWorkSt>"
  Bus Selector3/57 -> OMAPve_y_ADAS_SRR_RF_FCTAWrn/1, ob_convert100/1  "<OMAPve_y_ADAS_SRR_RF_FCTAWrn>"
  OMAPve_y_ADAS_L0LineType_2/1 -> ob_convert182/1
  OMAPve_y_ADAS_L1LineType_2/1 -> ob_convert183/1
  OMAPve_y_ADAS_R0LineType_2/1 -> ob_convert184/1
  OMAPve_y_ADAS_R1LineType_2/1 -> ob_convert185/1
  OMAPve_y_ADAS_LineCurveType_2/1 -> ob_convert186/1
  OMAPve_y_ADAS_FrontObject01Zone_2/1 -> ob_convert187/1
  OMAPve_y_ADAS_FrontObj01Class_2/1 -> ob_convert188/1
  OMAPve_y_ADAS_FrontObject02Zone_2/1 -> ob_convert189/1
  OMAPve_y_ADAS_FrontObj02Class_2/1 -> ob_convert190/1
  OMAPve_y_ADAS_FrontObject03Zone_2/1 -> ob_convert191/1
  OMAPve_y_ADAS_FrontObj03Class_2/1 -> ob_convert192/1
  OMAPve_y_ADAS_FrontObject04Zone_2/1 -> ob_convert193/1
  OMAPve_y_ADAS_FrontObj04Class_2/1 -> ob_convert194/1
  OMAPve_y_ADAS_FrontObject05Zone_2/1 -> ob_convert195/1
  OMAPve_y_ADAS_FrontObj05Class_2/1 -> ob_convert196/1
  OMAPve_y_ADAS_FrontObject06Zone_2/1 -> ob_convert197/1
  OMAPve_y_ADAS_FrontObj06Class_2/1 -> ob_convert198/1
  OMAPve_y_ADAS_BackObjectLeft_2/1 -> ob_convert199/1
  OMAPve_y_ADAS_BackObjectRight_2/1 -> ob_convert200/1
  OMAPve_y_ADAS_L0_LINE_TYPE_2/1 -> ob_convert202/1
  OMAPve_g_ADAS_L0_C0_COEF_2/1 -> ob_convert201/1
  OMAPve_g_ADAS_L0_C1_COEF_2/1 -> ob_convert203/1
  OMAPve_g_ADAS_L0_C2_COEF_2/1 -> ob_convert204/1
  OMAPve_g_ADAS_L0_C3_COEF_2/1 -> ob_convert205/1
  OMAPve_y_ADAS_R0_LINE_TYPE_2/1 -> ob_convert207/1
  OMAPve_g_ADAS_R0_C0_COEF_2/1 -> ob_convert206/1
  OMAPve_g_ADAS_R0_C1_COEF_2/1 -> ob_convert208/1
  OMAPve_g_ADAS_R0_C2_COEF_2/1 -> ob_convert209/1
  OMAPve_g_ADAS_R0_C3_COEF_2/1 -> ob_convert210/1
  OMAPve_g_ADAS_OBJ01_LatDis_2/1 -> ob_convert211/1
  OMAPve_g_ADAS_OBJ01_LgtDis_2/1 -> ob_convert212/1
  OMAPve_y_ADAS_OBJ01_Class_2/1 -> ob_convert213/1
  OMAPve_y_ADAS_OBJ01_ID_2/1 -> ob_convert214/1
  OMAPve_y_ADAS_OBJ01_Lane_2/1 -> ob_convert216/1
  OMAPve_g_ADAS_OBJ02_LatDis_2/1 -> ob_convert215/1
  OMAPve_g_ADAS_OBJ02_LgtDis_2/1 -> ob_convert217/1
  OMAPve_y_ADAS_OBJ02_Class_2/1 -> ob_convert218/1
  OMAPve_y_ADAS_OBJ02_ID_2/1 -> ob_convert219/1
  OMAPve_y_ADAS_OBJ02_Lane_2/1 -> ob_convert221/1
  OMAPve_g_ADAS_OBJ03_LatDis_2/1 -> ob_convert220/1
  OMAPve_g_ADAS_OBJ03_LgtDis_2/1 -> ob_convert222/1
  OMAPve_y_ADAS_OBJ03_Class_2/1 -> ob_convert223/1
  OMAPve_y_ADAS_OBJ03_ID_2/1 -> ob_convert224/1
  OMAPve_y_ADAS_OBJ03_Lane_2/1 -> ob_convert226/1
  OMAPve_g_ADAS_OBJ04_LatDis_2/1 -> ob_convert225/1
  OMAPve_g_ADAS_OBJ04_LgtDis_2/1 -> ob_convert227/1
  OMAPve_y_ADAS_OBJ04_Class_2/1 -> ob_convert228/1
  OMAPve_y_ADAS_OBJ04_ID_2/1 -> ob_convert229/1
  OMAPve_y_ADAS_OBJ04_Lane_2/1 -> ob_convert231/1
  OMAPve_g_ADAS_OBJ05_LatDis_2/1 -> ob_convert230/1
  OMAPve_g_ADAS_OBJ05_LgtDis_2/1 -> ob_convert232/1
  OMAPve_y_ADAS_OBJ05_Class_2/1 -> ob_convert233/1
  OMAPve_y_ADAS_OBJ05_ID_2/1 -> ob_convert234/1
  OMAPve_y_ADAS_OBJ05_Lane_2/1 -> ob_convert236/1
  OMAPve_g_ADAS_OBJ06_LatDis_2/1 -> ob_convert235/1
  OMAPve_g_ADAS_OBJ06_LgtDis_2/1 -> ob_convert237/1
  OMAPve_y_ADAS_OBJ06_Class_2/1 -> ob_convert238/1
  OMAPve_y_ADAS_OBJ06_ID_2/1 -> ob_convert239/1
  OMAPve_y_ADAS_OBJ06_Lane_2/1 -> ob_convert240/1
  AEBS_Direct/5(AEB_Input) -> [AEB_Input]
  Bus Selector3/3 -> OMAPve_y_ADAS_ISASignType/1, ob_convert3/1  "<OMAPve_y_ISA_Sign_Type_2>"
  Bus Selector3/4 -> OMAPve_y_ADAS_ISAStatus/1, ob_convert4/1  "<OMAPve_y_ISA_Status_2>"
  AEBS_Direct/3(AEB_EPS) -> [AEB_EPS]
  Bus Selector3/29 -> OMAPve_y_ADAS_ICAMassageDisp/1, ob_convert56/1  "<OMAPve_y_ICA_HMI_Txt_Disp_2>"
  Bus Selector1/11 -> Terminator5/1  "<OMAPve_y_FCW_Status_1>"
  [AEB_IC] -> Index Vector3/5
  EW_ISA_TSR_Direct/1(EW_ISA_TSR_EMS) -> [EW_ISA_TSR_EMS]
  Bus Selector/6 -> Terminator3/1  "<OMAPve_y_stAcvTqWhlPTPotReq_1>"
  ICA_Direct_G59/3(ICA_Input) -> [ICA_Input]
  [EW_ISA_TSR_EMS] -> Index Vector/11
  Bus Selector/4 -> OMAPve_y_ADAS_TorqueActivReq/1, ob_convert24/1  "<OMAPve_y_Powertrain_torquewheel_request_1>"
  Bus Selector/2 -> Terminator2/1  "<OMAPve_g_PotACCTqReq_1>"
  ELKS_Direct/3(ELK_EPS) -> [ELK_EPS]
  [LKA_EMS] -> Index Vector/7
  [EW_ISA_TSR_EPS] -> Index Vector2/11
  Default_EMS/1(Default_EMS) -> Index Vector/3, Index Vector/12, Index Vector/2
  [LKA_EPS] -> Index Vector2/7
  Index Vector4/1 -> Bus Selector4/1
  ICA_Direct_G59/2(ICA_IC) -> [ICA_IC]
  [ELK_IC] -> Index Vector3/8
  Bus Selector3/6 -> OMAPve_y_ADAS_ACCHeadwayDisplay/1, ob_convert8/1  "<OMAPve_y_ACC_DesiredHeadway_Display_2>"
  Bus Selector1/3 -> OMAPve_y_ADAS_PrefillRequest/1, ob_convert30/1  "<OMAPve_y_Prefill_request_1>"
  EW_ISA_TSR_Direct/4(EW_ISA_TSR_IC) -> [EW_ISA_TSR_IC]
  [ELK_EMS] -> Index Vector/8
  Default_OTHER/1(Default) -> Index Vector4/4, Index Vector4/2
  Constant/1 -> Index Vector/1  "Switch_EMS"
  ELKS_Direct/4(ELK_IC) -> [ELK_IC]
  AEBS_Direct/4(AEB_IC) -> [AEB_IC]
  Bus Selector3/17 -> OMAPve_y_ADAS_HMITargetDispFlag/1, ob_convert19/1  "<OMAPve_y_ACC_HMI_TgtDisp_Flag_2>"
  Bus Selector3/16 -> OMAPve_y_ADAS_AEBMassageDisp/1, ob_convert18/1  "<OMAPve_y_AEB_tips_2>"
  EW_ISA_TSR_Direct/5(EW_Input) -> [EW_Input]
  [JA_EPS] -> Index Vector2/6
  Constant4/1 -> Index Vector4/1  "Switch"
  AEBS_Direct/2(AEB_ESC) -> [AEB_ESC]
  Bus Selector4/3 -> OMAPve_y_ADAS_UpDownGearChange/1, ob_convert26/1  "<OMAPve_y_TYPE_RAPPORT_2>"
  [FD_Input] -> LKAS_Direct/2(Input_FDMM)
  [ELK_EPS] -> Index Vector2/8
  LKAS_Direct/1(LKA_EMS) -> [LKA_EMS]
  LKAS_Direct/3(LKA_EPS) -> [LKA_EPS]
  [AEB_EPS] -> Index Vector2/5
  [ACC_EPS] -> Index Vector2/4
  ESAS_Direct/4(ESA_IC) -> [ESA_IC]
  Bus Selector3/23 -> OMAPve_y_ADAS_LDWStatusDisplay/1, ob_convert42/1  "<OMAPve_y_LDW_Status_Display_2>"
  Bus Selector3/25 -> OMAPve_y_ADAS_LKAStatusDisplay/1, ob_convert44/1  "<OMAPve_y_LKA_Status_Display_2>"
  Bus Selector2/5 -> OMAPve_y_ADAS_LKAActivation/1, ob_convert52/1  "<OMAPve_y_Permit_to_know_if_LKA_or_LPA3F2_2>"
  Bus Selector3/26 -> OMAPve_y_ADAS_LKASwitchState/1, ob_convert45/1  "<OMAPve_y_LKA_Switch_State_2>"
  Bus Selector2/4 -> OMAPve_g_ADAS_LKAAngleReq/1, ob_convert51/1  "<OMAPve_g_Column_angle_setpoint3F2_2>"
  Bus Selector2/3 -> OMAPve_g_ADAS_LKATorqFactReq/1, ob_convert50/1  "<OMAPve_g_Coefficient_toregulate_EPS_2>"
  [ESA_EPS] -> Index Vector2/9
  Bus Selector3/7 -> OMAPve_y_ADAS_ACCHeadwayIcon/1, ob_convert9/1  "<OMAPve_y_ACC_DesiredHeadway_Icon_Basic_2>"
  Bus Selector1/6 -> OMAPve_y_ADAS_DecelerationType/1, ob_convert33/1  "<OMAPve_y_MDD_deceleration_type_1>"
  Default_ESC/1(Default_ESC) -> Index Vector1/3, Index Vector1/12, Index Vector1/2
  Bus Selector1/7 -> Terminator4/1  "<OMAPve_y_State_of_the_functionFARC_det_1>"
  Bus Selector3/10 -> OMAPve_y_ADAS_ACCStatusIconDis/1, ob_convert12/1  "<OMAPve_y_ACC_Vehicle_Icon_Display_2>"
  Bus Selector3/30 -> OMAPve_y_ADAS_ICAStatusIcon/1, ob_convert57/1  "<OMAPve_y_TJA_status_icon_2>"
  [ESA_EMS] -> Index Vector/9
  Bus Selector3/2 -> OMAPve_y_ADAS_ISAPopupMessage/1, ob_convert2/1  "<OMAPve_y_ISA_Popup_text_2>"
  ACCS_Direct/6(ACC_to_ICA) -> [ACC_to_ICA]
  [AEB_ESC] -> Index Vector1/5
  ACCS_Direct/1(ACC_EMS) -> [ACC_EMS]
  Bus Selector3/24 -> OMAPve_y_ADAS_LKAMode/1, ob_convert43/1  "<OMAPve_y_LKA_Mode_from_Camera_2>"
  Default_EPS/1(Default_EPS) -> Index Vector2/3, Index Vector2/12, Index Vector2/2
  [JA_IC] -> Index Vector3/6
  [FD_Input] -> ESAS_Direct/2(Input_FDMM)
  Bus Selector4/2 -> Terminator9/1  "<OMAPve_y_ASR_connection_dis_demand2_2>"
  Bus Selector3/18 -> OMAPve_y_ADAS_TargetPosition/1, ob_convert20/1  "<OMAPve_y_TARGET_POSITION_2>"
  JABS_Direct/1(JA_EMS) -> [JA_EMS]
  [FD_Input] -> ELKS_Direct/2(Input_FDMM)
  [ACC_ESC] -> [ICA_ESC]
  Bus Selector/1 -> Terminator1/1  "<OMAPve_y_ACC_Engine_Start_Request_1>"
  Bus Selector3/27 -> Terminator7/1  "<OMAPve_y_LKA_action_indication_2>"
  Constant1/1 -> Index Vector1/1  "Switch_ESC"
  Bus Selector3/21 -> OMAPve_y_ADAS_VehicleLaneDisp/1, ob_convert40/1  "<OMAPve_y_Vehicle_Lane_Display_2>"
  ESAS_Direct/1(ESA_EMS) -> [ESA_EMS]
  Bus Selector1/8 -> OMAPve_y_ADAS_AEBState/1, ob_convert34/1  "<OMAPve_y_AEB_Status_1>"
  [ACC_EMS] -> Index Vector/4
  Bus Selector3/9 -> OMAPve_y_ADAS_ACCSetSpeedDis/1, ob_convert11/1  "<OMAPve_y_ACC_Set_Speed_Display_2>"
  Bus Selector2/1 -> Terminator6/1  "<OMAPve_y_Power_steering_power_cut3F2_2>"
  ACCS_Direct/4(ACC_IC) -> [ACC_IC]
  Bus Selector/5 -> OMAPve_g_ADAS_DownorUpGearMinTime/1, ob_convert25/1  "<OMAPve_g_TminUp_or_downGear_1>"
  OMAPve_y_Dead_man_dedicated_push_button2Num/1 -> Terminator10/1
  Bus Selector1/12 -> OMAPve_y_ADAS_HapticAlarmReq/1, ob_convert37/1  "<OMAPve_y_Haptic_Alarm_1>"
  ELKS_Direct/1(ELK_EMS) -> [ELK_EMS]
  Bus Selector/7 -> OMAPve_y_ADAS_ACCState/1, ob_convert27/1  "<OMAPve_y_Function_Acc_status_1>"
  [ACC_EMS] -> [ICA_EMS]
  JABS_Direct/4(JA_IC) -> [JA_IC]
  Bus Selector1/9 -> OMAPve_y_ADAS_BrakeRequest/1, ob_convert35/1  "<OMAPve_y_Decel_Request_1>"
  [ESA_IC] -> Index Vector3/9
  JABS_Direct/2(JA_ESC) -> [JA_ESC]
  [JA_ESC] -> Index Vector1/6
  Bus Selector3/12 -> OMAPve_y_ADAS_ACCMessagePrompt/1, ob_convert14/1  "<OMAPve_y_ACC_Pop_Up_Message_2>"
  [AEB_EMS] -> Index Vector/5
  Bus Selector4/4 -> OMAPve_y_ADAS_OperatingStatus/1, ob_convert63/1  "<OMAPve_y_ECU_operating_phase_2>"
  Bus Selector1/2 -> OMAPve_y_ADAS_DeclControlReq/1, ob_convert29/1  "<OMAPve_y_MDD_Decelerationcontrol_request_1>"
  Bus Selector4/1 -> Terminator8/1  "<OMAPve_y_ABS_ESP_power_cut_request2_2>"
  Bus Selector3/14 -> OMAPve_y_ADAS_AEBFaultStatus/1, ob_convert16/1  "<OMAPve_y_AEB_Fault_Status_2>"
  Bus Selector1/10 -> OMAPve_y_ADAS_AEBBrakingProg/1, ob_convert36/1  "<OMAPve_y_AEB_Braking_progress_1>"
  [ICA_EMS] -> Index Vector/10
  [ACC_ESC] -> Index Vector1/4
  ELKS_Direct/5(ELK_Input) -> [ELK_Input]
  Bus Selector3/15 -> OMAPve_y_ADAS_AEBSwitchStatus/1, ob_convert17/1  "<OMAPve_y_AEB_Switch_Status_2>"
  LKAS_Direct/5(LKA_Input) -> [LKA_Input]
  [JA_EMS] -> Index Vector/6
  ESAS_Direct/3(ESA_EPS) -> [ESA_EPS]
  Bus Selector1/1 -> OMAPve_g_ADAS_DecelerationSet/1, ob_convert28/1  "<OMAPve_g_Deceleration_setpoint_device_1>"
  [ICA_ESC] -> Index Vector1/10
  OMAPve_y_EASYMOVE_powercut_request3F2Num/1 -> Terminator11/1
  Bus Selector3/11 -> OMAPve_y_ADAS_ACC_RVVReqType/1, ob_convert13/1  "<OMAPve_y_RVVACC_Vehiclespeed_request_type_2>"
  LKAS_Direct/2(LKA_ESC) -> [LKA_ESC]
  ICA_Direct_G59/1(ICA_EPS) -> [ICA_EPS]
  Default_IC/1(Default_IC) -> Index Vector3/3, Index Vector3/12, Index Vector3/2
  Bus Selector4/5 -> OMAPve_y_ADAS_Radar_State/1, ob_convert66/1  "<OMAPve_y_Radar_State_2>"
  JABS_Direct/3(JA_EPS) -> [JA_EPS]
  Bus Selector3/19 -> OMAPve_y_ADAS_Handsoffwarning/1, ob_convert38/1  "<OMAPve_y_Hands_off_warning_2>"
  AEBS_Direct/1(AEB_EMS) -> [AEB_EMS]
  ELKS_Direct/2(ELK_ESC) -> [ELK_ESC]
  JABS_Direct/5(JA_Input) -> [JA_Input]
  ACCS_Direct/3(ACC_EPS) -> [ACC_EPS]
  Bus Selector3/22 -> OMAPve_y_ADAS_LDWWarningSt/1, ob_convert41/1  "<OMAPve_y_LDW_Flag_2>"
  [EW_ISA_TSR_IC] -> Index Vector3/11
  Bus Selector3/5 -> OMAPve_y_ADAS_ISAValue/1, ob_convert5/1  "<OMAPve_y_ISA_Value_2>"
  Constant3/1 -> Index Vector3/1  "Switch_IC"
  [ELK_ESC] -> Index Vector1/8
  [ESA_ESC] -> Index Vector1/9
  Bus Selector3/8 -> OMAPve_y_ADAS_ACCSetSpeed/1, ob_convert10/1  "<OMAPve_y_ACC_Desired_Set_Speed_2>"
  Index Vector1/1 -> Bus Selector1/1
  Index Vector/1 -> Bus Selector/1
  Constant6/1 -> Terminator/1  "ob_OMAP_version"
  [ACC_IC] -> Index Vector3/4
  ACCS_Direct/5(ACC_Input) -> [ACC_Input]
  LKAS_Direct/4(LKA_IC) -> [LKA_IC]
  EW_ISA_TSR_Direct/2(EW_ISA_TSR_ESC) -> [EW_ISA_TSR_ESC]
  [EW_ISA_TSR_ESC] -> Index Vector1/11
  Index Vector3/1 -> Bus Selector3/1
  EW_ISA_TSR_Direct/3(EW_ISA_TSR_EPS) -> [EW_ISA_TSR_EPS]
  Bus Selector3/20 -> OMAPve_y_ADAS_HMIPopupMassage/1, ob_convert39/1  "<OMAPve_y_HMI_Popup_Status_2>"
  [LKA_ESC] -> Index Vector1/7
  Bus Selector3/13 -> OMAPve_y_ADAS_AEBAlertReq/1, ob_convert15/1  "<OMAPve_y_AEB_Alert_Req_2>"
  ACCS_Direct/2(ACC_ESC) -> [ACC_ESC]
  OMAPve_y_Trailer_Present3F2Num/1 -> Terminator12/1
  Index Vector2/1 -> Bus Selector2/1
  Bus Selector3/1 -> OMAPve_y_ADAS_TSRSignType/1, ob_convert1/1  "<OMAPve_y_TSR_Vision_Only_Sign_Type_2>"
  ESAS_Direct/2(ESA_ESC) -> [ESA_ESC]
  Bus Selector/3 -> OMAPve_g_ADAS_ACCTorqueReq/1, ob_convert23/1  "<OMAPve_g_ACCTqReq_1>"
  Bus Selector2/2 -> OMAPve_y_ADAS_LKAState/1, ob_convert49/1  "<OMAPve_y_General_state_of_LKA_function3F2_2>"
  Constant2/1 -> Index Vector2/1  "Switch_EPS"
  [LKA_IC] -> Index Vector3/7
  [ICA_IC] -> Index Vector3/10
  OTHER_Default_Arbitration/1(Arbitration) -> Index Vector4/3
  Bus Selector3/28 -> OMAPve_y_ADAS_ELKSts/1, ob_convert46/1  "<OMAPve_y_ADAS_ELKSts_2>"
  Bus Selector1/5 -> OMAPve_y_ADAS_ESCHoldReq/1, ob_convert32/1  "<OMAPve_y_ADAS_ESCHoldReq>"
  Bus Selector1/4 -> OMAPve_y_ADAS_ESCDriveOff/1, ob_convert31/1  "<OMAPve_y_ADAS_ESCDriveOff>"
  Bus Selector1/13 -> OMAPve_y_ADAS_ACCRequestEPB/1, ob_convert67/1  "<OMAPve_y_ADAS_ACCRequestEPB>"
  Bus Selector3/31 -> OMAPve_y_ADAS_SRR_SystemState/1, ob_convert74/1  "<OMAPve_y_ADAS_SRR_SystemState>"
  Bus Selector3/32 -> OMAPve_y_ADAS_LeftLEDWarningSt/1, ob_convert75/1  "<OMAPve_y_ADAS_LeftLEDWarningSt>"
  Bus Selector3/33 -> OMAPve_y_ADAS_RighrLEDWarningSt/1, ob_convert76/1  "<OMAPve_y_ADAS_RighrLEDWarningSt>"
  Bus Selector3/36 -> OMAPve_y_ADAS_BSD_ErrorSt/1, ob_convert79/1  "<OMAPve_y_ADAS_BSD_ErrorSt>"
  Bus Selector3/37 -> OMAPve_y_ADAS_BSD_LCAWarning/1, ob_convert80/1  "<OMAPve_y_ADAS_BSD_LCAWarning>"
  Bus Selector3/38 -> OMAPve_y_ADAS_BSD_DoorOpenWrn/1, ob_convert81/1  "<OMAPve_y_ADAS_BSD_DoorOpenWrn>"
  Bus Selector3/39 -> OMAPve_y_ADAS_BSD_RCTAWarning/1, ob_convert82/1  "<OMAPve_y_ADAS_BSD_RCTAWarning>"
  Bus Selector3/40 -> OMAPve_y_ADAS_BSD_DOWWorkingSt/1, ob_convert83/1  "<OMAPve_y_ADAS_BSD_DOWWorkingSt>"
  Bus Selector3/41 -> OMAPve_y_ADAS_BSD_RCTAWorkingSt/1, ob_convert84/1  "<OMAPve_y_ADAS_BSD_RCTAWorkingSt>"
  Bus Selector3/42 -> OMAPve_y_ADAS_BSD_S_SystStInfo/1, ob_convert85/1  "<OMAPve_y_ADAS_BSD_S_SystStInfo>"
  Bus Selector3/43 -> OMAPve_y_ADAS_BSD_S_LCWWorkSt/1, ob_convert86/1  "<OMAPve_y_ADAS_BSD_S_LCWWorkSt>"
  Bus Selector3/44 -> OMAPve_y_ADAS_BSD_S_ErrorSt/1, ob_convert87/1  "<OMAPve_y_ADAS_BSD_S_ErrorSt>"
  Bus Selector3/45 -> OMAPve_y_ADAS_BSD_S_LCAWarning/1, ob_convert88/1  "<OMAPve_y_ADAS_BSD_S_LCAWarning>"
  Bus Selector3/52 -> OMAPve_y_ADAS_SRR_LF_ErrorSt/1, ob_convert95/1  "<OMAPve_y_ADAS_SRR-LF_ErrorSt>"
  Bus Selector3/53 -> OMAPve_y_ADAS_SRR_LF_FCTAWrn/1, ob_convert96/1  "<OMAPve_y_ADAS_SRR_LF_FCTAWrn>"
  Bus Selector3/54 -> OMAPve_y_ADAS_SRR_RF_SystStInfo/1, ob_convert97/1  "<OMAPve_y_ADAS_SRR_RF_SystStInfo>"
  Bus Selector3/55 -> OMAPve_y_ADAS_SRR_RF_SystWorkSt/1, ob_convert98/1  "<OMAPve_y_ADAS_SRR_RF_SystWorkSt>"
  Bus Selector3/56 -> OMAPve_y_ADAS_SRR_RF_ErrorSt/1, ob_convert99/1  "<OMAPve_y_ADAS_SRR-RF_ErrorSt>"
  Bus Selector3/49 -> OMAPve_y_ADAS_BSD_S_RCTAWorkSt/1, ob_convert92/1  "<OMAPve_y_ADAS_BSD_S_RCTAWorkSt>"
  Bus Selector3/48 -> OMAPve_y_ADAS_BSD_S_DOWWorkSt/1, ob_convert91/1  "<OMAPve_y_ADAS_BSD_S_DOWWorkSt>"
  Bus Selector3/47 -> OMAPve_y_ADAS_BSD_S_RCTAWarning/1, ob_convert90/1  "<OMAPve_y_ADAS_BSD_S_RCTAWarning>"
  ob_convert1/1 -> ob_terminator1/1  "ob_OMAPve_y_ADAS_TSRSignType"
  ob_convert2/1 -> ob_terminator2/1  "ob_OMAPve_y_ADAS_ISAPopupMsg"
  ob_convert3/1 -> ob_terminator3/1  "ob_OMAPve_y_ADAS_ISASignType"
  ob_convert4/1 -> ob_terminator4/1  "ob_OMAPve_y_ADAS_ISAStatus"
  ob_convert5/1 -> ob_terminator5/1  "ob_OMAPve_y_ADAS_ISAValue"
  ob_convert6/1 -> ob_terminator6/1  "ob_OMAPve_y_ADAS_ISLCState"
  ob_convert7/1 -> ob_terminator7/1  "ob_OMAPve_y_ADAS_ISLCDriverRmd"
  ob_convert8/1 -> ob_terminator8/1  "ob_OMAPve_y_ADAS_ACCHeadwayDisp"
  ob_convert9/1 -> ob_terminator9/1  "ob_OMAPve_y_ADAS_ACCHeadwayIcon"
  ob_convert10/1 -> ob_terminator10/1  "ob_OMAPve_y_ADAS_ACCSetSpeed"
  ob_convert11/1 -> ob_terminator11/1  "ob_OMAPve_y_ADAS_ACCSetSpeedDis"
  ob_convert12/1 -> ob_terminator12/1  "ob_OMAPve_y_ADAS_ACCStIconDis"
  ob_convert13/1 -> ob_terminator13/1  "ob_OMAPve_y_ADAS_ACC_RVVReqType"
  ob_convert14/1 -> ob_terminator14/1  "ob_OMAPve_y_ADAS_ACCMsgPrompt"
  ob_convert15/1 -> ob_terminator15/1  "ob_OMAPve_y_ADAS_AEBAlertReq"
  ob_convert16/1 -> ob_terminator16/1  "ob_OMAPve_y_ADAS_AEBFaultStatus"
  ob_convert17/1 -> ob_terminator17/1  "ob_OMAPve_y_ADAS_AEBSwitchSt"
  ob_convert18/1 -> ob_terminator18/1  "ob_OMAPve_y_ADAS_AEBMassageDisp"
  ob_convert19/1 -> ob_terminator19/1  "ob_OMAPve_y_ADAS_HMITargDispFlg"
  ob_convert20/1 -> ob_terminator20/1  "ob_OMAPve_y_ADAS_TargetPosition"
  ob_convert21/1 -> ob_terminator21/1  "ob_OMAPve_y_ADAS_ACCLongiDist"
  ob_convert22/1 -> ob_terminator22/1  "ob_OMAPve_y_ADAS_ACCLateralDist"
  ob_convert23/1 -> ob_terminator23/1  "ob_OMAPve_g_ADAS_ACCTorqueReq"
  ob_convert24/1 -> ob_terminator24/1  "ob_OMAPve_y_ADAS_TorqueActivReq"
  ob_convert25/1 -> ob_terminator25/1  "ob_OMAPve_g_ADAS_DownUpMinTime"
  ob_convert26/1 -> ob_terminator26/1  "ob_OMAPve_y_ADAS_UpDownGearCng"
  ob_convert27/1 -> ob_terminator27/1  "ob_OMAPve_y_ADAS_ACCState"
  ob_convert28/1 -> ob_terminator28/1  "ob_OMAPve_g_ADAS_DecelSet"
  ob_convert29/1 -> ob_terminator29/1  "ob_OMAPve_y_ADAS_DeclControlReq"
  ob_convert30/1 -> ob_terminator30/1  "ob_OMAPve_y_ADAS_PrefillRequest"
  ob_convert31/1 -> ob_terminator31/1  "ob_OMAPve_y_ADAS_ESCDriveOff"
  ob_convert32/1 -> ob_terminator32/1  "ob_OMAPve_y_ADAS_ESCHoldReq"
  ob_convert33/1 -> ob_terminator33/1  "ob_OMAPve_y_ADAS_DecelType"
  ob_convert34/1 -> ob_terminator34/1  "ob_OMAPve_y_ADAS_AEBState"
  ob_convert35/1 -> ob_terminator35/1  "ob_OMAPve_y_ADAS_BrakeRequest"
  ob_convert36/1 -> ob_terminator36/1  "ob_OMAPve_y_ADAS_AEBBrakingProg"
  ob_convert37/1 -> ob_terminator37/1  "ob_OMAPve_y_ADAS_HapticAlarmReq"
  ob_convert38/1 -> ob_terminator38/1  "ob_OMAPve_y_ADAS_Handsoffwarn"
  ob_convert39/1 -> ob_terminator39/1  "ob_OMAPve_y_ADAS_HMIPopupMsg"
  ob_convert40/1 -> ob_terminator40/1  "ob_OMAPve_y_ADAS_VehicleLaneDis"
  ob_convert41/1 -> ob_terminator41/1  "ob_OMAPve_y_ADAS_LDWWarningSt"
  ob_convert42/1 -> ob_terminator42/1  "ob_OMAPve_y_ADAS_LDWStatusDisp"
  ob_convert43/1 -> ob_terminator43/1  "ob_OMAPve_y_ADAS_LKAMode"
  ob_convert44/1 -> ob_terminator44/1  "ob_OMAPve_y_ADAS_LKAStatusDisp"
  ob_convert45/1 -> ob_terminator45/1  "ob_OMAPve_y_ADAS_LKASwitchState"
  ob_convert46/1 -> ob_terminator46/1  "ob_OMAPve_y_ADAS_ELKSts"
  ob_convert47/1 -> ob_terminator47/1  "ob_OMAPve_y_ADAS_LCAStatusDisp"
  ob_convert48/1 -> ob_terminator48/1  "ob_OMAPve_y_ADAS_LCAPopupMsg"
  ob_convert49/1 -> ob_terminator49/1  "ob_OMAPve_y_ADAS_LKAState"
  ob_convert50/1 -> ob_terminator50/1  "ob_OMAPve_g_ADAS_LKATorqFactReq"
  ob_convert51/1 -> ob_terminator51/1  "ob_OMAPve_g_ADAS_LKAAngleReq"
  ob_convert52/1 -> ob_terminator52/1  "ob_OMAPve_y_ADAS_LKAActivation"
  ob_convert53/1 -> ob_terminator53/1  "ob_OMAPve_y_ADAS_ESAState"
  ob_convert54/1 -> ob_terminator54/1  "ob_OMAPve_g_ADAS_ESATorqueReq"
  ob_convert55/1 -> ob_terminator55/1  "ob_OMAPve_y_ADAS_ESARequest"
  ob_convert56/1 -> ob_terminator56/1  "ob_OMAPve_y_ADAS_ICAMassageDisp"
  ob_convert57/1 -> ob_terminator57/1  "ob_OMAPve_y_ADAS_ICAStatusIcon"
  ob_convert58/1 -> ob_terminator58/1  "ob_OMAPve_y_ADAS_HWAMode"
  ob_convert59/1 -> ob_terminator59/1  "ob_OMAPve_y_ADAS_HWATurnOnIdctr"
  ob_convert60/1 -> ob_terminator60/1  "ob_OMAPve_y_ADAS_ESAFaultSt"
  ob_convert61/1 -> ob_terminator61/1  "ob_OMAPve_y_ADAS_JAFaultSt"
  ob_convert62/1 -> ob_terminator62/1  "ob_OMAPve_y_ADAS_HWAActionSts"
  ob_convert63/1 -> ob_terminator63/1  "ob_OMAPve_y_ADAS_OperatingSt"
  ob_convert64/1 -> ob_terminator64/1  "ob_OMAPve_y_ADAS_IHBC_HB_Req"
  ob_convert65/1 -> ob_terminator65/1  "ob_OMAPve_y_ADAS_IHBC_FuctionSt"
  ob_convert66/1 -> ob_terminator66/1  "ob_OMAPve_y_ADAS_Radar_State"
  ob_convert67/1 -> ob_terminator67/1  "ob_OMAPve_y_ADAS_ACCRequestEPB"
  ob_convert68/1 -> ob_terminator68/1  "ob_OMAPve_y_ADAS_EngStartReqSTT"
  ob_convert69/1 -> ob_terminator69/1  "ob_OMAPve_y_ADAS_EngStopPmtSTT"
  ob_convert70/1 -> ob_terminator70/1  "ob_OMAPve_y_ADAS_State"
  ob_convert71/1 -> ob_terminator71/1  "ob_OMAPve_y_ADAS_LetfLigthCtrl"
  ob_convert72/1 -> ob_terminator72/1  "ob_OMAPve_y_ADAS_RightLigthCtrl"
  ob_convert73/1 -> ob_terminator73/1  "ob_OMAPve_y_ADAS_LightCtrlValid"
  ob_convert74/1 -> ob_terminator74/1  "ob_OMAPve_y_ADAS_SRR_SystemSt"
  ob_convert75/1 -> ob_terminator75/1  "ob_OMAPve_y_ADAS_LeftLEDWarnSt"
  ob_convert76/1 -> ob_terminator76/1  "ob_OMAPve_y_ADAS_RighrLEDWarnSt"
  ob_convert77/1 -> ob_terminator77/1  "ob_OMAPve_y_ADAS_BSDSysStInfo"
  ob_convert78/1 -> ob_terminator78/1  "ob_OMAPve_y_ADAS_BSDLCWWorkSt"
  ob_convert79/1 -> ob_terminator79/1  "ob_OMAPve_y_ADAS_BSD_ErrorSt"
  ob_convert80/1 -> ob_terminator80/1  "ob_OMAPve_y_ADAS_BSD_LCAWarning"
  ob_convert81/1 -> ob_terminator81/1  "ob_OMAPve_y_ADAS_BSDDoorOpenWrn"
  ob_convert82/1 -> ob_terminator82/1  "ob_OMAPve_y_ADAS_BSDRCTAWarning"
  ob_convert83/1 -> ob_terminator83/1  "ob_OMAPve_y_ADAS_BSD_DOWWorkSt"
  ob_convert84/1 -> ob_terminator84/1  "ob_OMAPve_y_ADAS_BSD_RCTAWorkSt"
  ob_convert85/1 -> ob_terminator85/1  "ob_OMAPve_y_ADAS_BSDS_SysStInfo"
  ob_convert86/1 -> ob_terminator86/1  "ob_OMAPve_y_ADAS_BSDS_LCWWorkSt"
  ob_convert87/1 -> ob_terminator87/1  "ob_OMAPve_y_ADAS_BSD_S_ErrorSt"
  ob_convert88/1 -> ob_terminator88/1  "ob_OMAPve_y_ADAS_BSD_S_LCAWarn"
  ob_convert89/1 -> ob_terminator89/1  "ob_OMAPve_y_ADAS_BSDSDoorOpenWn"
  ob_convert90/1 -> ob_terminator90/1  "ob_OMAPve_y_ADAS_BSD_S_RCTAWarn"
  ob_convert91/1 -> ob_terminator91/1  "ob_OMAPve_y_ADAS_BSDS_DOWWorkSt"
  ob_convert92/1 -> ob_terminator92/1  "ob_OMAPve_y_ADAS_BSDSRCTAWorkSt"
  ob_convert93/1 -> ob_terminator93/1  "ob_OMAPve_y_ADAS_SRRLFSysStInfo"
  ob_convert94/1 -> ob_terminator94/1  "ob_OMAPve_y_ADAS_SRRLFSysWorkSt"
  ob_convert95/1 -> ob_terminator95/1  "ob_OMAPve_y_ADAS_SRR_LF_ErrorSt"
  ob_convert96/1 -> ob_terminator96/1  "ob_OMAPve_y_ADAS_SRR_LF_FCTAWrn"
  ob_convert97/1 -> ob_terminator97/1  "ob_OMAPve_y_ADAS_SRRRFSysStInfo"
  ob_convert98/1 -> ob_terminator98/1  "ob_OMAPve_y_ADAS_SRRRFSysWorkSt"
  ob_convert99/1 -> ob_terminator99/1  "ob_OMAPve_y_ADAS_SRR_RF_ErrorSt"
  ob_convert100/1 -> ob_terminator100/1  "ob_OMAPve_y_ADAS_SRR_RF_FCTAWrn"
  ob_convert101/1 -> ob_terminator101/1  "ob_OMAPve_y_ADAS_L0LineType"
  ob_convert102/1 -> ob_terminator102/1  "ob_OMAPve_y_ADAS_L1LineType"
  ob_convert103/1 -> ob_terminator103/1  "ob_OMAPve_y_ADAS_R0LineType"
  ob_convert104/1 -> ob_terminator104/1  "ob_OMAPve_y_ADAS_R1LineType"
  ob_convert105/1 -> ob_terminator105/1  "ob_OMAPve_y_ADAS_LineCurveType"
  ob_convert106/1 -> ob_terminator106/1  "ob_OMAPve_y_ADAS_FrontObj01Zone"
  ob_convert107/1 -> ob_terminator107/1  "ob_OMAPve_y_ADAS_FrtObj01Class"
  ob_convert108/1 -> ob_terminator108/1  "ob_OMAPve_y_ADAS_FrontObj02Zone"
  ob_convert109/1 -> ob_terminator109/1  "ob_OMAPve_y_ADAS_FrtObj02Class"
  ob_convert110/1 -> ob_terminator110/1  "ob_OMAPve_y_ADAS_FrontOb03Zone"
  ob_convert111/1 -> ob_terminator111/1  "ob_OMAPve_y_ADAS_FrtObj03Class"
  ob_convert112/1 -> ob_terminator112/1  "ob_OMAPve_y_ADAS_FrontObj04Zone"
  ob_convert113/1 -> ob_terminator113/1  "ob_OMAPve_y_ADAS_FrtObj04Class"
  ob_convert114/1 -> ob_terminator114/1  "ob_OMAPve_y_ADAS_FrontObj05Zone"
  ob_convert115/1 -> ob_terminator115/1  "ob_OMAPve_y_ADAS_FrtObj05Class"
  ob_convert116/1 -> ob_terminator116/1  "ob_OMAPve_y_ADAS_FrontObj06Zone"
  ob_convert117/1 -> ob_terminator117/1  "ob_OMAPve_y_ADAS_FrtObj06Class"
  ob_convert118/1 -> ob_terminator118/1  "ob_OMAPve_y_ADAS_BackObjectLeft"
  ob_convert119/1 -> ob_terminator119/1  "ob_OMAPve_y_ADAS_BackObjRight"
  ob_convert120/1 -> ob_terminator120/1  "ob_OMAPve_y_ADAS_L0_LINE_TYPE"
  ob_convert121/1 -> ob_terminator121/1  "ob_OMAPve_g_ADAS_L0_C0_COEF"
  ob_convert122/1 -> ob_terminator122/1  "ob_OMAPve_g_ADAS_L0_C1_COEF"
  ob_convert123/1 -> ob_terminator123/1  "ob_OMAPve_g_ADAS_L0_C2_COEF"
  ob_convert124/1 -> ob_terminator124/1  "ob_OMAPve_g_ADAS_L0_C3_COEF"
  ob_convert125/1 -> ob_terminator125/1  "ob_OMAPve_y_ADAS_R0_LINE_TYPE"
  ob_convert126/1 -> ob_terminator126/1  "ob_OMAPve_g_ADAS_R0_C0_COEF"
  ob_convert127/1 -> ob_terminator127/1  "ob_OMAPve_g_ADAS_R0_C1_COEF"
  ob_convert128/1 -> ob_terminator128/1  "ob_OMAPve_g_ADAS_R0_C2_COEF"
  ob_convert129/1 -> ob_terminator129/1  "ob_OMAPve_g_ADAS_R0_C3_COEF"
  ob_convert130/1 -> ob_terminator130/1  "ob_OMAPve_g_ADAS_OBJ01_LatDis"
  ob_convert131/1 -> ob_terminator131/1  "ob_OMAPve_g_ADAS_OBJ01_LgtDis"
  ob_convert132/1 -> ob_terminator132/1  "ob_OMAPve_y_ADAS_OBJ01_Class"
  ob_convert133/1 -> ob_terminator133/1  "ob_OMAPve_y_ADAS_OBJ01_ID"
  ob_convert134/1 -> ob_terminator134/1  "ob_OMAPve_y_ADAS_OBJ01_Lane"
  ob_convert135/1 -> ob_terminator135/1  "ob_OMAPve_g_ADAS_OBJ02_LatDis"
  ob_convert136/1 -> ob_terminator136/1  "ob_OMAPve_g_ADAS_OBJ02_LgtDis"
  ob_convert137/1 -> ob_terminator137/1  "ob_OMAPve_y_ADAS_OBJ02_Class"
  ob_convert138/1 -> ob_terminator138/1  "ob_OMAPve_y_ADAS_OBJ02_ID"
  ob_convert139/1 -> ob_terminator139/1  "ob_OMAPve_y_ADAS_OBJ02_Lane"
  ob_convert140/1 -> ob_terminator140/1  "ob_OMAPve_g_ADAS_OBJ03_LatDis"
  ob_convert141/1 -> ob_terminator141/1  "ob_OMAPve_g_ADAS_OBJ03_LgtDis"
  ob_convert142/1 -> ob_terminator142/1  "ob_OMAPve_y_ADAS_OBJ03_Class"
  ob_convert143/1 -> ob_terminator143/1  "ob_OMAPve_y_ADAS_OBJ03_ID"
  ob_convert144/1 -> ob_terminator144/1  "ob_OMAPve_y_ADAS_OBJ03_Lane"
  ob_convert145/1 -> ob_terminator145/1  "ob_OMAPve_g_ADAS_OBJ04_LatDis"
  ob_convert146/1 -> ob_terminator146/1  "ob_OMAPve_g_ADAS_OBJ04_LgtDis"
  ob_convert147/1 -> ob_terminator147/1  "ob_OMAPve_y_ADAS_OBJ04_Class"
  ob_convert148/1 -> ob_terminator148/1  "ob_OMAPve_y_ADAS_OBJ04_ID"
  ob_convert149/1 -> ob_terminator149/1  "ob_OMAPve_y_ADAS_OBJ04_Lane"
  ob_convert150/1 -> ob_terminator150/1  "ob_OMAPve_g_ADAS_OBJ05_LatDis"
  ob_convert151/1 -> ob_terminator151/1  "ob_OMAPve_g_ADAS_OBJ05_LgtDis"
  ob_convert152/1 -> ob_terminator152/1  "ob_OMAPve_y_ADAS_OBJ05_Class"
  ob_convert153/1 -> ob_terminator153/1  "ob_OMAPve_y_ADAS_OBJ05_ID"
  ob_convert154/1 -> ob_terminator154/1  "ob_OMAPve_y_ADAS_OBJ05_Lane"
  ob_convert155/1 -> ob_terminator155/1  "ob_OMAPve_g_ADAS_OBJ06_LatDis"
  ob_convert156/1 -> ob_terminator156/1  "ob_OMAPve_g_ADAS_OBJ06_LgtDis"
  ob_convert157/1 -> ob_terminator157/1  "ob_OMAPve_y_ADAS_OBJ06_Class"
  ob_convert158/1 -> ob_terminator158/1  "ob_OMAPve_y_ADAS_OBJ06_ID"
  ob_convert159/1 -> ob_terminator159/1  "ob_OMAPve_y_ADAS_OBJ06_Lane"
  ob_convert160/1 -> OMAPve_y_ADAS_ISLCState/1, ob_convert6/1
  ob_convert161/1 -> OMAPve_y_ADAS_ISLCDriverRemind/1, ob_convert7/1
  ob_convert162/1 -> OMAPve_y_ADAS_ACCLongiDist/1, ob_convert21/1
  ob_convert163/1 -> OMAPve_y_ADAS_ACCLateralDist/1, ob_convert22/1
  ob_convert164/1 -> OMAPve_y_ADAS_LCAStatusDisplay/1, ob_convert47/1
  ob_convert165/1 -> OMAPve_y_ADAS_LCAPopupMessage/1, ob_convert48/1
  ob_convert166/1 -> OMAPve_y_ADAS_ESAState/1, ob_convert53/1
  ob_convert167/1 -> OMAPve_y_ADAS_ESARequest/1, ob_convert55/1
  ob_convert168/1 -> OMAPve_g_ADAS_ESATorqueReq/1, ob_convert54/1
  ob_convert169/1 -> OMAPve_y_ADAS_HWAMode/1, ob_convert58/1
  ob_convert170/1 -> OMAPve_y_ADAS_HWATurnOnIdctr/1, ob_convert59/1
  ob_convert171/1 -> OMAPve_y_ADAS_ESAFaultSt/1, ob_convert60/1
  ob_convert172/1 -> OMAPve_y_ADAS_JAFaultSt/1, ob_convert61/1
  ob_convert173/1 -> OMAPve_y_ADAS_HWAActionSts/1, ob_convert62/1
  ob_convert174/1 -> OMAPve_y_ADAS_IHBC_HB_Req/1, ob_convert64/1
  ob_convert175/1 -> OMAPve_y_ADAS_IHBC_Fuction_St/1, ob_convert65/1
  ob_convert176/1 -> OMAPve_y_ADAS_EngStartReqForSTT/1, ob_convert68/1
  ob_convert177/1 -> OMAPve_y_ADAS_EngStopPmtForSTT/1, ob_convert69/1
  ob_convert179/1 -> OMAPve_y_ADAS_LetfLigthControl/1, ob_convert71/1
  ob_convert180/1 -> OMAPve_y_ADAS_RightLigthControl/1, ob_convert72/1
  ob_convert181/1 -> OMAPve_y_ADAS_LightControlValid/1, ob_convert73/1
  ob_convert184/1 -> OMAPve_y_ADAS_R0LineType/1, ob_convert103/1
  ob_convert183/1 -> OMAPve_y_ADAS_L1LineType/1, ob_convert102/1
  ob_convert182/1 -> OMAPve_y_ADAS_L0LineType/1, ob_convert101/1
  ob_convert185/1 -> OMAPve_y_ADAS_R1LineType/1, ob_convert104/1
  ob_convert186/1 -> OMAPve_y_ADAS_LineCurveType/1, ob_convert105/1
  ob_convert187/1 -> OMAPve_y_ADAS_FrontObject01Zone/1, ob_convert106/1
  ob_convert188/1 -> OMAPve_y_ADAS_FrontObj01Class/1, ob_convert107/1
  ob_convert189/1 -> OMAPve_y_ADAS_FrontObject02Zone/1, ob_convert108/1
  ob_convert190/1 -> OMAPve_y_ADAS_FrontObj02Class/1, ob_convert109/1
  ob_convert193/1 -> OMAPve_y_ADAS_FrontObject04Zone/1, ob_convert112/1
  ob_convert191/1 -> OMAPve_y_ADAS_FrontObject03Zone/1, ob_convert110/1
  ob_convert192/1 -> OMAPve_y_ADAS_FrontObj03Class/1, ob_convert111/1
  ob_convert195/1 -> OMAPve_y_ADAS_FrontObject05Zone/1, ob_convert114/1
  ob_convert194/1 -> OMAPve_y_ADAS_FrontObj04Class/1, ob_convert113/1
  ob_convert196/1 -> OMAPve_y_ADAS_FrontObj05Class/1, ob_convert115/1
  ob_convert197/1 -> OMAPve_y_ADAS_FrontObject06Zone/1, ob_convert116/1
  ob_convert198/1 -> OMAPve_y_ADAS_FrontObj06Class/1, ob_convert117/1
  ob_convert199/1 -> OMAPve_y_ADAS_BackObjectLeft/1, ob_convert118/1
  ob_convert200/1 -> OMAPve_y_ADAS_BackObjectRight/1, ob_convert119/1
  ob_convert202/1 -> OMAPve_y_ADAS_L0_LINE_TYPE/1, ob_convert120/1
  ob_convert201/1 -> OMAPve_g_ADAS_L0_C0_COEF/1, ob_convert121/1
  ob_convert203/1 -> OMAPve_g_ADAS_L0_C1_COEF/1, ob_convert122/1
  ob_convert204/1 -> OMAPve_g_ADAS_L0_C2_COEF/1, ob_convert123/1
  ob_convert205/1 -> OMAPve_g_ADAS_L0_C3_COEF/1, ob_convert124/1
  ob_convert206/1 -> OMAPve_g_ADAS_R0_C0_COEF/1, ob_convert126/1
  ob_convert208/1 -> OMAPve_g_ADAS_R0_C1_COEF/1, ob_convert127/1
  ob_convert207/1 -> OMAPve_y_ADAS_R0_LINE_TYPE/1, ob_convert125/1
  ob_convert209/1 -> OMAPve_g_ADAS_R0_C2_COEF/1, ob_convert128/1
  ob_convert210/1 -> OMAPve_g_ADAS_R0_C3_COEF/1, ob_convert129/1
  ob_convert211/1 -> OMAPve_g_ADAS_OBJ01_LatDis/1, ob_convert130/1
  ob_convert212/1 -> OMAPve_g_ADAS_OBJ01_LgtDis/1, ob_convert131/1
  ob_convert213/1 -> OMAPve_y_ADAS_OBJ01_Class/1, ob_convert132/1
  ob_convert214/1 -> OMAPve_y_ADAS_OBJ01_ID/1, ob_convert133/1
  ob_convert215/1 -> OMAPve_g_ADAS_OBJ02_LatDis/1, ob_convert135/1
  ob_convert216/1 -> OMAPve_y_ADAS_OBJ01_Lane/1, ob_convert134/1
  ob_convert217/1 -> OMAPve_g_ADAS_OBJ02_LgtDis/1, ob_convert136/1
  ob_convert218/1 -> OMAPve_y_ADAS_OBJ02_Class/1, ob_convert137/1
  ob_convert219/1 -> OMAPve_y_ADAS_OBJ02_ID/1, ob_convert138/1
  ob_convert220/1 -> OMAPve_g_ADAS_OBJ03_LatDis/1, ob_convert140/1
  ob_convert221/1 -> OMAPve_y_ADAS_OBJ02_Lane/1, ob_convert139/1
  ob_convert223/1 -> OMAPve_y_ADAS_OBJ03_Class/1, ob_convert142/1
  ob_convert222/1 -> OMAPve_g_ADAS_OBJ03_LgtDis/1, ob_convert141/1
  ob_convert224/1 -> OMAPve_y_ADAS_OBJ03_ID/1, ob_convert143/1
  ob_convert225/1 -> OMAPve_g_ADAS_OBJ04_LatDis/1, ob_convert145/1
  ob_convert226/1 -> OMAPve_y_ADAS_OBJ03_Lane/1, ob_convert144/1
  ob_convert227/1 -> OMAPve_g_ADAS_OBJ04_LgtDis/1, ob_convert146/1
  ob_convert229/1 -> OMAPve_y_ADAS_OBJ04_ID/1, ob_convert148/1
  ob_convert228/1 -> OMAPve_y_ADAS_OBJ04_Class/1, ob_convert147/1
  ob_convert230/1 -> OMAPve_g_ADAS_OBJ05_LatDis/1, ob_convert150/1
  ob_convert232/1 -> OMAPve_g_ADAS_OBJ05_LgtDis/1, ob_convert151/1
  ob_convert233/1 -> OMAPve_y_ADAS_OBJ05_Class/1, ob_convert152/1
  ob_convert234/1 -> OMAPve_y_ADAS_OBJ05_ID/1, ob_convert153/1
  ob_convert231/1 -> OMAPve_y_ADAS_OBJ04_Lane/1, ob_convert149/1
  ob_convert235/1 -> OMAPve_g_ADAS_OBJ06_LatDis/1, ob_convert155/1
  ob_convert237/1 -> OMAPve_g_ADAS_OBJ06_LgtDis/1, ob_convert156/1
  ob_convert238/1 -> OMAPve_y_ADAS_OBJ06_Class/1, ob_convert157/1
  ob_convert236/1 -> OMAPve_y_ADAS_OBJ05_Lane/1, ob_convert154/1
  ob_convert239/1 -> OMAPve_y_ADAS_OBJ06_ID/1, ob_convert158/1
  ob_convert240/1 -> OMAPve_y_ADAS_OBJ06_Lane/1, ob_convert159/1
  ob_convert178/1 -> OMAPve_y_ADAS_State/1, ob_convert70/1
  Ground/1 -> ob_In_convert144/1, Data Type Conversion182/1
  Ground1/1 -> ob_In_convert143/1, Data Type Conversion180/1
  Data Type Conversion84/1 -> Bus_ACCS/18  "ACCSve_d_ACC_GoIndicateReq_LZM_convert"
  Data Type Conversion109/1 -> Bus_LKAS/10  "LKASve_g_EPS_Factor_Control_convert"
  Data Type Conversion175/1 -> Bus_JABS/13  "JABSve_d_DbTips_convert"
  Data Type Conversion177/1 -> Bus_JABS/15  "JABSve_d_DbESCHoldReq_convert"
  Data Type Conversion173/1 -> Bus_JABS/11  "JABSve_d_DbFltStatus_convert"
  ELKSve_g_EPS_Factor_Control/1 -> Data Type Conversion145/1, ob_In_convert83/1
  IMAPve_g_ESC_LonAcc/1 -> Data Type Conversion56/1, ob_In_convert118/1
  Data Type Conversion140/1 -> Bus_ELKS/3  "ELKSve_y_Hands_Off_Warning_convert"
  Data Type Conversion92/1 -> Bus_ACCS/4  "ACCSve_g_ACC_DecReq_convert"
  Data Type Conversion116/1 -> Bus_LKAS/3  "LKASve_y_LKA_Status_Display_convert"
  Data Type Conversion127/1 -> Bus_EW/8  "EWWWve_y_BSD_S_LCAWarning_convert"
  Data Type Conversion170/1 -> Bus_JABS/7  "JABSve_d_DbBraking_progress_convert"
  Data Type Conversion93/1 -> Bus_ACCS/3  "ACCSve_d_ACC_TqFlag_convert"
  Data Type Conversion56/1 -> Bus_IMAP/2  "IMAPve_g_ESC_LonAcc_convert"
  ELKSve_y_ELK_HapticAlarmReq/1 -> Data Type Conversion139/1, ob_In_convert77/1
  Data Type Conversion171/1 -> Bus_JABS/9  "JABSve_d_DbJACWStatus_convert"
  Data Type Conversion141/1 -> Bus_ELKS/4  "ELKSve_y_ELK_Action_Indication_convert"
  JABSve_d_DbTips/1 -> Data Type Conversion175/1, ob_In_convert62/1
  ACCSve_d_VelocitySet/1 -> Data Type Conversion62/1, ob_In_convert21/1
  Data Type Conversion132/1 -> Bus_EW/13  "EWWWve_y_SRR_LF_FCTAWarning_convert"
  Data Type Conversion169/1 -> Bus_JABS/6  "JABSve_d_DbHapticAlarm_convert"
  Data Type Conversion82/1 -> Bus_ACCS/16  "ACCSve_d_ACC_CtlVeh_LZM_convert"
  Data Type Conversion2/1 -> Bus_ACCS/14  "ACCSve_d_ACC_ESCHoldReq_convert"
  Data Type Conversion165/1 -> Bus_JABS/2  "JABSve_d_DbFunFARCSta_convert"
  JABSve_d_DbHapticAlarm/1 -> Data Type Conversion169/1, ob_In_convert55/1
  Data Type Conversion133/1 -> Bus_EW/14  "EWWWve_y_SRR_RF_FCTAWarning_convert"
  Data Type Conversion161/1 -> Bus_AEBS/3  "AEBSve_g_DecSetpoint_convert"
  FDMMve_d_SignalTStamp/1 -> Data Type Conversion21/1, ob_In_convert12/1
  ICADva_d_DecionState/1 -> Data Type Conversion27/1, ob_In_convert94/1
  Data Type Conversion147/1 -> Bus_ELKS/10  "ELKSve_y_ELK_VehicleLaneDisp_convert"
  Data Type Conversion158/1 -> Bus_AEBS/6  "AEBSve_d_ESCDriveOff_convert"
  Data Type Conversion58/1 -> Bus_FDMM/4  "FDMMve_d_ElkFcnConf_convert"
  AEBSve_d_JABS_FltStatus/1 -> Data Type Conversion6/1, ob_In_convert46/1
  Data Type Conversion154/1 -> Bus_AEBS/10  "AEBSve_d_AEBStatus_convert"
  Data Type Conversion150/1 -> Bus_AEBS/14  "AEBSve_d_AEBAlertReq_convert"
  Data Type Conversion121/1 -> Bus_EW/2  "EWWWve_y_RCTA_M_SystemWorkingSt_convert"
  Data Type Conversion145/1 -> Bus_ELKS/8  "ELKSve_g_EPS_Factor_Control_convert"
  IMAPve_g_R0_C0/1 -> Data Type Conversion105/1, ob_In_convert126/1
  Data Type Conversion163/1 -> Bus_AEBS/1  "AEBSve_d_Prefill_request_convert"
  Ground5/1 -> ob_In_convert139/1, Data Type Conversion87/1
  Data Type Conversion160/1 -> Bus_AEBS/4  "AEBSve_d_MDDdecRequest_convert"
  Data Type Conversion95/1 -> Bus_ACCS/1  "ACCSve_d_ACC_State_convert"
  Data Type Conversion128/1 -> Bus_EW/9  "EWWWve_y_BSD_S_DoorOpenWarning_convert"
  JABSve_d_DbFunFARCSta/1 -> Data Type Conversion165/1, ob_In_convert51/1
  ELKSve_y_EPS_ELK_Control/1 -> Data Type Conversion146/1, ob_In_convert84/1
  Data Type Conversion162/1 -> Bus_AEBS/2  "AEBSve_d_functionFARCState_convert"
  Data Type Conversion155/1 -> Bus_AEBS/9  "AEBSve_d_Braking_progress_convert"
  AEBSve_d_AEBSwitchStatus/1 -> Data Type Conversion152/1, ob_In_convert39/1
  Data Type Conversion79/1 -> Bus_AEBS/24  "AEBSve_d_DAS1_Status_DBS_Enable_convert"
  Data Type Conversion21/1 -> Bus_FDMM/12  "FDMMve_d_SignalTStamp_convert"
  ACCSve_d_ACC_ESCHoldReq/1 -> Data Type Conversion2/1, ob_In_convert26/1
  AEBSve_d_JABS_HapticAlarm/1 -> Data Type Conversion5/1, ob_In_convert48/1
  JABSve_d_DbJACWStatus/1 -> Data Type Conversion171/1, ob_In_convert58/1
  Ground8/1 -> ob_In_convert136/1, Data Type Conversion79/1
  Data Type Conversion182/1 -> Bus_ICA/8  "ICABve_g_LKATorqueReq_Value_convert"
  Data Type Conversion148/1 -> Bus_ELKS/11  "ELKSve_y_ELK_ELKSts_convert"
  Data Type Conversion135/1 -> Bus_EW/16  "EWWWve_y_BSD_S_SystemStateInfo_convert"
  EWWWve_y_BSD_S_SystemStateInfo/1 -> Data Type Conversion135/1, ob_In_convert113/1
  IMAPve_d_ESC_Veh_Standstill/1 -> Data Type Conversion100/1, ob_In_convert121/1
  JABSve_d_DbSignalTStamp/1 -> Data Type Conversion30/1, ob_In_convert57/1
  Data Type Conversion178/1 -> Bus_ELKS/13  "ELKSve_y_LKATorqueReq_convert"
  Data Type Conversion151/1 -> Bus_AEBS/13  "AEBSve_d_AEBFaultStatus_convert"
  Ground11/1 -> ob_In_convert131/1, Data Type Conversion83/1
  Ground13/1 -> ob_In_convert133/1, Data Type Conversion85/1
  ACCSve_d_ACC_go_request/1 -> Data Type Conversion63/1, ob_In_convert20/1
  ACCSve_d_SignalTStamp/1 -> Data Type Conversion3/1, ob_In_convert23/1
  AEBSve_d_ESCDriveOff/1 -> Data Type Conversion158/1, ob_In_convert33/1
  ACCSve_d_ACC_EPBReq/1 -> Data Type Conversion/1, ob_In_convert27/1
  LKASve_y_LKA_Status_Display/1 -> Data Type Conversion116/1, ob_In_convert67/1
  Data Type Conversion180/1 -> Bus_ICA/7  "ICABve_d_LKATorqueReq_convert"
  JABSve_d_DbPrefillReq/1 -> Data Type Conversion164/1, ob_In_convert50/1
  LKASve_g_LKA_SWA_Control/1 -> Data Type Conversion110/1, ob_In_convert73/1
  Data Type Conversion23/1 -> Bus_ICA/1  "ICABva_d_PathQI_convert"
  AEBSve_d_AEBAlertReq/1 -> Data Type Conversion150/1, ob_In_convert41/1
  Data Type Conversion15/1 -> Bus_FDMM/9  "FDMMve_d_AlcFcnConf_convert"
  ACCSve_d_ACC_ESCDriveOff/1 -> Data Type Conversion1/1, ob_In_convert25/1
  Data Type Conversion172/1 -> Bus_JABS/10  "JABSve_d_DbSwitchStatus_convert"
  JABSve_d_DbAlertReq/1 -> Data Type Conversion174/1, ob_In_convert61/1
  Ground14/1 -> ob_In_convert134/1, Data Type Conversion86/1
  Data Type Conversion27/1 -> Bus_ICA/9  "ICADva_d_DecionState_convert"
  ICADva_d_DecionCMD/1 -> Data Type Conversion26/1, ob_In_convert95/1
  IMAPve_g_R0_C2/1 -> Data Type Conversion107/1, ob_In_convert128/1
  Ground7/1 -> ob_In_convert137/1, Data Type Conversion80/1
  Data Type Conversion112/1 -> Bus_LKAS/7  "LKASve_y_HMI_Popup_Status_convert"
  LKASve_y_EPS_LKA_Control/1 -> Data Type Conversion119/1, ob_In_convert75/1
  Ground3/1 -> ob_In_convert141/1, Data Type Conversion178/1
  Ground12/1 -> ob_In_convert132/1, Data Type Conversion84/1
  Data Type Conversion89/1 -> Bus_ACCS/7  "ACCSve_d_ACCActive_Signal_convert"
  Data Type Conversion102/1 -> Bus_IMAP/7  "IMAPve_g_L0_C1_convert"
  Data Type Conversion157/1 -> Bus_AEBS/7  "AEBSve_d_ESCHoldReq_convert"
  ELKSve_g_ELK_SWA_Control/1 -> Data Type Conversion144/1, ob_In_convert82/1
  Data Type Conversion98/1 -> Bus_IMAP/3  "IMAPva_d_obj_id_convert"
  Data Type Conversion91/1 -> Bus_ACCS/5  "ACCSve_d_ACC_DecFlag_convert"
  AEBSve_d_HapticAlarm/1 -> Data Type Conversion156/1, ob_In_convert35/1
  Data Type Conversion96/1 -> Bus_ACCS/12  "ACCSve_d_ACC_ICA_Flag_convert"
  Data Type Conversion62/1 -> Bus_ACCS/9  "ACCSve_d_VelocitySet_convert"
  Data Type Conversion20/1 -> Bus_FDMM/8  "FDMMve_d_LfFcnConf_convert"
  ICABve_d_ICAState/1 -> Data Type Conversion24/1, ob_In_convert93/1
  Data Type Conversion54/1 -> Bus_ICA/4  "ICABve_g_SteerAngleCmd_convert"
  ELKSve_y_SignalTStamp/1 -> Data Type Conversion11/1, ob_In_convert87/1
  Data Type Conversion57/1 -> Bus_FDMM/5  "FDMMve_d_LkaFcnConf_convert"
  EWWWve_y_LCW_M_SystemWorkingSt/1 -> Data Type Conversion120/1, ob_In_convert98/1
  Data Type Conversion83/1 -> Bus_ACCS/17  "ACCSve_d_ACC_CancelReq_LZM_convert"
  Data Type Conversion85/1 -> Bus_ACCS/19  "ACCSve_d_ACC_OverrideIndReq_LZM_convert"
  Data Type Conversion86/1 -> Bus_ACCS/20  "AACCSve_d_ACC_TakeoverIndReq_LZM_convert"
  IMAPve_d_EPS_LKA_State/1 -> Data Type Conversion97/1, ob_In_convert117/1
  FDMMve_g_Adas2Fapa/1 -> Data Type Conversion22/1, ob_In_convert11/1
  AEBSve_d_AEBTips/1 -> Data Type Conversion149/1, ob_In_convert42/1
  Data Type Conversion87/1 -> Bus_LKAS/12  "LKASve_y_LKATorqueReq_convert"
  Data Type Conversion179/1 -> Bus_ELKS/14  "ELKSve_g_LKATorqueReq_Value_convert"
  FDMMve_d_LfFcnConf/1 -> Data Type Conversion20/1, ob_In_convert8/1
  Ground4/1 -> ob_In_convert140/1, Data Type Conversion88/1
  Data Type Conversion78/1 -> Bus_AEBS/23  "AEBSve_d_DAS1_Status_AEBJerkWarning_Lvl_convert"
  AEBSve_d_Prefill_request/1 -> Data Type Conversion163/1, ob_In_convert28/1
  ELKSve_y_Hands_Off_Warning/1 -> Data Type Conversion140/1, ob_In_convert78/1
  ELKSve_y_EPS_State_Control/1 -> Data Type Conversion143/1, ob_In_convert81/1
  AEBSve_d_Braking_progress/1 -> Data Type Conversion155/1, ob_In_convert36/1
  Data Type Conversion168/1 -> Bus_JABS/5  "JABSve_d_DbMDDdecType_convert"
  ACCSve_g_ACC_TqReq/1 -> Data Type Conversion94/1, ob_In_convert14/1
  ICABve_d_SignalTStamp/1 -> Data Type Conversion25/1, ob_In_convert89/1
  AEBSve_d_JABS_AlertSign/1 -> Data Type Conversion7/1, ob_In_convert44/1
  Bus_ACCS/1 -> ACCS_Direct/1(Input_ACCS)  "Input_ACCS"
  IMAPve_g_L0_C3/1 -> Data Type Conversion104/1, ob_In_convert125/1
  ELKSve_y_ELK_Action_Indication/1 -> Data Type Conversion141/1, ob_In_convert79/1
  ICABve_d_ICAMode/1 -> Data Type Conversion55/1, ob_In_convert92/1
  Data Type Conversion28/1 -> Bus_ICA/11  "ICADva_d_LCRecommend_convert"
  ELKSve_y_HMI_Popup_Status/1 -> Data Type Conversion142/1, ob_In_convert80/1
  Data Type Conversion11/1 -> Bus_ELKS/12  "ELKSve_y_SignalTStamp_convert"
  IMAPve_g_R0_C3/1 -> Data Type Conversion108/1, ob_In_convert129/1
  FDMMve_d_ElkFcnConf/1 -> Data Type Conversion58/1, ob_In_convert4/1
  LKASve_y_EPS_State_Control/1 -> Data Type Conversion111/1, ob_In_convert72/1
  LKASve_y_HMI_Popup_Status/1 -> Data Type Conversion112/1, ob_In_convert71/1
  Data Type Conversion55/1 -> Bus_ICA/5  "ICABve_d_ICAMode_convert"
  FDMMve_d_JaFcnConf/1 -> Data Type Conversion19/1, ob_In_convert1/1
  AEBSve_d_functionFARCState/1 -> Data Type Conversion162/1, ob_In_convert29/1
  IMAPva_g_obj_pos_x/1 -> Data Type Conversion99/1, ob_In_convert120/1
  FDMMve_d_EwFcnConf/1 -> Data Type Conversion17/1, ob_In_convert10/1
  IMAPve_g_L0_C0/1 -> Data Type Conversion101/1, ob_In_convert122/1
  JABSve_d_DbBraking_progress/1 -> Data Type Conversion170/1, ob_In_convert56/1
  Data Type Conversion16/1 -> Bus_FDMM/3  "FDMMve_d_EsaFcnConf_convert"
  ACCSve_d_ACC_DecFlag/1 -> Data Type Conversion91/1, ob_In_convert17/1
  AEBSve_d_ESCHoldReq/1 -> Data Type Conversion157/1, ob_In_convert34/1
  Data Type Conversion26/1 -> Bus_ICA/10  "ICADva_d_DecionCMD_convert"
  Data Type Conversion99/1 -> Bus_IMAP/4  "IMAPva_g_obj_pos_x_convert"
  Data Type Conversion149/1 -> Bus_AEBS/15  "AEBSve_d_AEBTips_convert"
  ELKSve_y_state_ELK_function/1 -> Data Type Conversion12/1, ob_In_convert76/1
  LKASve_y_LKA_Action_Indication/1 -> Data Type Conversion113/1, ob_In_convert70/1
  ACCSve_d_ACC_ICA_Flag/1 -> Data Type Conversion96/1, ob_In_convert24/1
  Data Type Conversion22/1 -> Bus_FDMM/11  "FDMMve_g_Adas2Fapa_convert"
  FDMMve_d_EsaFcnConf/1 -> Data Type Conversion16/1, ob_In_convert3/1
  Data Type Conversion6/1 -> Bus_AEBS/19  "AEBSve_d_JABS_FltStatus_convert"
  Data Type Conversion174/1 -> Bus_JABS/12  "JABSve_d_DbAlertReq_convert"
  ACCSve_d_ACCActive_Signal/1 -> Data Type Conversion89/1, ob_In_convert19/1
  EWWWve_y_BSD_S_DoorOpenWarning/1 -> Data Type Conversion128/1, ob_In_convert106/1
  Data Type Conversion159/1 -> Bus_AEBS/5  "AEBSve_d_MDDdecType_convert"
  Data Type Conversion9/1 -> Bus_AEBS/22  "AEBSve_d_JABS_Tips_convert"
  AEBSve_g_DecSetpoint/1 -> Data Type Conversion161/1, ob_In_convert30/1
  FDMMve_d_AccFcnConf/1 -> Data Type Conversion13/1, ob_In_convert7/1
  ICADve_d_SignalTStamp/1 -> Data Type Conversion29/1, ob_In_convert97/1
  ACCSve_d_CIPV_ID/1 -> Data Type Conversion90/1, ob_In_convert18/1
  Data Type Conversion126/1 -> Bus_EW/7  "EWWWve_y_BSD_M_RCTAWarning_convert"
  EWWWve_y_SRR_SystemState/1 -> Data Type Conversion134/1, ob_In_convert112/1
  FDMMve_d_LkaFcnConf/1 -> Data Type Conversion57/1, ob_In_convert5/1
  EWWWve_y_DOW_M_SystemWorkingSt/1 -> Data Type Conversion122/1, ob_In_convert100/1
  JABSve_d_DbESCHoldReq/1 -> Data Type Conversion177/1, ob_In_convert64/1
  IMAPve_g_L0_C1/1 -> Data Type Conversion102/1, ob_In_convert123/1
  Data Type Conversion/1 -> Bus_ACCS/15  "ACCSve_d_ACC_EPBReq_convert"
  Data Type Conversion13/1 -> Bus_FDMM/7  "FDMMve_d_AccFcnConf_convert"
  Data Type Conversion17/1 -> Bus_FDMM/10  "FDMMve_d_EwFcnConf_convert"
  FDMMve_d_IcaFcnConf/1 -> Data Type Conversion18/1, ob_In_convert6/1
  Data Type Conversion24/1 -> Bus_ICA/6  "ICABve_d_ICAState_convert"
  Data Type Conversion25/1 -> Bus_ICA/2  "ICABve_d_SignalTStamp_convert"
  Data Type Conversion18/1 -> Bus_FDMM/6  "FDMMve_d_IcaFcnConf_convert"
  AEBSve_d_JABS_Tips/1 -> Data Type Conversion9/1, ob_In_convert49/1
  Data Type Conversion4/1 -> Bus_AEBS/20  "AEBSve_d_JABS_AlertReq_convert"
  LKASve_g_EPS_Factor_Control/1 -> Data Type Conversion109/1, ob_In_convert74/1
  ACCSve_d_HeadWaySet/1 -> Data Type Conversion60/1, ob_In_convert22/1
  AEBSve_d_AEBStatus/1 -> Data Type Conversion154/1, ob_In_convert37/1
  Data Type Conversion60/1 -> Bus_ACCS/10  "ACCSve_d_HeadWaySet_convert"
  Data Type Conversion146/1 -> Bus_ELKS/9  "ELKSve_y_EPS_ELK_Control_convert"
  Data Type Conversion139/1 -> Bus_ELKS/2  "ELKSve_y_ELK_HapticAlarmReq_convert"
  Data Type Conversion90/1 -> Bus_ACCS/6  "ACCSve_d_CIPV_ID_convert"
  Data Type Conversion166/1 -> Bus_JABS/3  "JABSve_g_DbDecSetpoint_convert"
  Data Type Conversion136/1 -> Bus_EW/17  "EWWWve_y_BSD_SystemStateInfo_convert"
  ACCSve_d_ACC_TqFlag/1 -> Data Type Conversion93/1, ob_In_convert15/1
  Data Type Conversion137/1 -> Bus_EW/18  "EWWWve_y_SRR_LF_SystemStateInfo_convert"
  Data Type Conversion138/1 -> Bus_EW/19  "EWWWve_y_SRR_RF_SystemStateInfo_convert"
  ACCSve_d_ACC_State/1 -> Data Type Conversion95/1, ob_In_convert13/1
  Data Type Conversion129/1 -> Bus_EW/10  "EWWWve_y_BSD_S_RCTAWarning_convert"
  EWWWve_y_SRR_RF_FCTAWarning/1 -> Data Type Conversion133/1, ob_In_convert111/1
  Data Type Conversion153/1 -> Bus_AEBS/11  "AEBSve_d_FCWStatus_convert"
  Data Type Conversion105/1 -> Bus_IMAP/10  "IMAPve_g_R0_C0_convert"
  Data Type Conversion130/1 -> Bus_EW/11  "EWWWve_y_SRR_LF_FCTAWorkingSt_convert"
  Data Type Conversion125/1 -> Bus_EW/6  "EWWWve_y_BSD_M_DoorOpenWarning_convert"
  Data Type Conversion122/1 -> Bus_EW/3  "EWWWve_y_DOW_M_SystemWorkingSt_convert"
  Data Type Conversion124/1 -> Bus_EW/5  "EWWWve_y_BSD_M_LCAWarning_convert"
  Data Type Conversion123/1 -> Bus_EW/4  "EWWWve_y_BSD_M_ErrorSt_convert"
  EWWWve_y_SRR_RF_SystemStateInfo/1 -> Data Type Conversion138/1, ob_In_convert116/1
  Data Type Conversion30/1 -> Bus_JABS/8  "JABSve_d_DbSignalTStamp_convert"
  Data Type Conversion118/1 -> Bus_LKAS/1  "LKASve_y_Vehicle_Lane_Display_convert"
  Data Type Conversion101/1 -> Bus_IMAP/6  "IMAPve_g_L0_C0_convert"
  LKASve_y_LDW_Status_Display/1 -> Data Type Conversion117/1, ob_In_convert66/1
  ACCSve_g_ACC_DecReq/1 -> Data Type Conversion92/1, ob_In_convert16/1
  Data Type Conversion142/1 -> Bus_ELKS/5  "ELKSve_y_HMI_Popup_Status_convert"
  Data Type Conversion97/1 -> Bus_IMAP/1  "IMAPve_d_EPS_LKA_State_convert"
  Data Type Conversion119/1 -> Bus_LKAS/11  "LKASve_y_EPS_LKA_Control_convert"
  EWWWve_y_BSD_SystemStateInfo/1 -> Data Type Conversion136/1, ob_In_convert114/1
  EWWWve_y_SRR_LF_ErrorSt/1 -> Data Type Conversion131/1, ob_In_convert109/1
  Data Type Conversion100/1 -> Bus_IMAP/5  "IMAPve_d_ESC_Veh_Standstill_convert"
  Data Type Conversion117/1 -> Bus_LKAS/2  "LKASve_y_LDW_Status_Display_convert"
  Data Type Conversion120/1 -> Bus_EW/1  "EWWWve_y_LCW_M_SystemWorkingSt_convert"
  LKASve_y_Hands_Off_Warning/1 -> Data Type Conversion114/1, ob_In_convert69/1
  Data Type Conversion115/1 -> Bus_LKAS/4  "LKASve_y_LDW_Flag_convert"
  Data Type Conversion19/1 -> Bus_FDMM/1  "FDMMve_d_JaFcnConf_convert"
  JABSve_d_DbMDDdecType/1 -> Data Type Conversion168/1, ob_In_convert54/1
  Data Type Conversion111/1 -> Bus_LKAS/8  "LKASve_y_EPS_State_Control_convert"
  AEBSve_d_JABS_SwitchStatus/1 -> Data Type Conversion8/1, ob_In_convert45/1
  EWWWve_y_BSD_M_LCAWarning/1 -> Data Type Conversion124/1, ob_In_convert102/1
  Data Type Conversion7/1 -> Bus_AEBS/17  "AEBSve_d_JABS_AlertSign_convert"
  Data Type Conversion107/1 -> Bus_IMAP/12  "IMAPve_g_R0_C2_convert"
  Data Type Conversion167/1 -> Bus_JABS/4  "JABSve_d_DbMDDdecRequest_convert"
  Data Type Conversion88/1 -> Bus_LKAS/13  "LKASve_g_LKATorqueReq_Value_convert"
  Data Type Conversion29/1 -> Bus_ICA/12  "ICADve_d_SignalTStamp_convert"
  AEBSve_d_FCWStatus/1 -> Data Type Conversion153/1, ob_In_convert38/1
  Ground6/1 -> ob_In_convert138/1, Data Type Conversion81/1
  AEBSve_d_SignalTStamp/1 -> Data Type Conversion10/1, ob_In_convert43/1
  Data Type Conversion176/1 -> Bus_JABS/14  "JABSve_d_DbESCDriveOff_convert"
  ELKSve_y_ELK_VehicleLaneDisp/1 -> Data Type Conversion147/1, ob_In_convert85/1
  AEBSve_d_JABS_AlertReq/1 -> Data Type Conversion4/1, ob_In_convert47/1
  EWWWve_y_BSD_M_ErrorSt/1 -> Data Type Conversion123/1, ob_In_convert101/1
  Data Type Conversion14/1 -> Bus_FDMM/2  "FDMMve_d_AebFcnConf_convert"
  JABSve_d_DbMDDdecRequest/1 -> Data Type Conversion167/1, ob_In_convert53/1
  EWWWve_y_SRR_LF_FCTAWarning/1 -> Data Type Conversion132/1, ob_In_convert110/1
  EWWWve_y_BSD_S_LCAWarning/1 -> Data Type Conversion127/1, ob_In_convert105/1
  EWWWve_y_SRR_LF_FCTAWorkingSt/1 -> Data Type Conversion130/1, ob_In_convert108/1
  IMAPva_d_obj_id/1 -> Data Type Conversion98/1, ob_In_convert119/1
  IMAPve_g_R0_C1/1 -> Data Type Conversion106/1, ob_In_convert127/1
  AEBSve_d_MDDdecType/1 -> Data Type Conversion159/1, ob_In_convert32/1
  Data Type Conversion10/1 -> Bus_AEBS/16  "AEBSve_d_SignalTStamp_convert"
  Ground2/1 -> ob_In_convert142/1, Data Type Conversion179/1
  Data Type Conversion113/1 -> Bus_LKAS/6  "LKASve_y_LKA_Action_Indication_convert"
  EWWWve_y_SRR_LF_SystemStateInfo/1 -> Data Type Conversion137/1, ob_In_convert115/1
  EWWWve_y_BSD_M_DoorOpenWarning/1 -> Data Type Conversion125/1, ob_In_convert103/1
  Data Type Conversion110/1 -> Bus_LKAS/9  "LKASve_g_LKA_SWA_Control_convert"
  JABSve_g_DbDecSetpoint/1 -> Data Type Conversion166/1, ob_In_convert52/1
  Data Type Conversion156/1 -> Bus_AEBS/8  "AEBSve_d_HapticAlarm_convert"
  Data Type Conversion1/1 -> Bus_ACCS/13  "ACCSve_d_ACC_ESCDriveOff_convert"
  JABSve_d_DbSwitchStatus/1 -> Data Type Conversion172/1, ob_In_convert59/1
  FDMMve_d_AebFcnConf/1 -> Data Type Conversion14/1, ob_In_convert2/1
  AEBSve_d_MDDdecRequest/1 -> Data Type Conversion160/1, ob_In_convert31/1
  Data Type Conversion144/1 -> Bus_ELKS/7  "ELKSve_g_ELK_SWA_Control_convert"
  ICABve_g_SteerAngleCmd/1 -> Data Type Conversion54/1, ob_In_convert91/1
  EWWWve_y_BSD_S_RCTAWarning/1 -> Data Type Conversion129/1, ob_In_convert107/1
  ICADva_d_LCRecommend/1 -> Data Type Conversion28/1, ob_In_convert96/1
  IMAPve_g_L0_C2/1 -> Data Type Conversion103/1, ob_In_convert124/1
  Bus Creator/1 -> ESAS_Direct/1(Input_ESAS), [ESA_Input]  "Input_ESAS"
  ICABva_d_PathQI/1 -> Data Type Conversion23/1, ob_In_convert88/1
  FDMMve_d_AlcFcnConf/1 -> Data Type Conversion15/1, ob_In_convert9/1
  JABSve_d_DbESCDriveOff/1 -> Data Type Conversion176/1, ob_In_convert63/1
  AEBSve_d_AEBFaultStatus/1 -> Data Type Conversion151/1, ob_In_convert40/1
  Data Type Conversion103/1 -> Bus_IMAP/8  "IMAPve_g_L0_C2_convert"
  ELKSve_y_ELK_ELKSts/1 -> Data Type Conversion148/1, ob_In_convert86/1
  EWWWve_y_BSD_M_RCTAWarning/1 -> Data Type Conversion126/1, ob_In_convert104/1
  Data Type Conversion8/1 -> Bus_AEBS/18  "AEBSve_d_JABS_SwitchStatus_convert"
  Data Type Conversion63/1 -> Bus_ACCS/8  "ACCSve_d_ACC_go_request_convert"
  Data Type Conversion143/1 -> Bus_ELKS/6  "ELKSve_y_EPS_State_Control_convert"
  LKASve_y_LDW_Flag/1 -> Data Type Conversion115/1, ob_In_convert68/1
  Data Type Conversion114/1 -> Bus_LKAS/5  "LKASve_y_Hands_Off_Warning_convert"
  Data Type Conversion3/1 -> Bus_ACCS/11  "ACCSve_d_SignalTStamp_convert"
  Bus_FDMM/1 -> [FD_Input]  "Input_FDMM"
  Data Type Conversion108/1 -> Bus_IMAP/13  "IMAPve_g_R0_C3_convert"
  Data Type Conversion152/1 -> Bus_AEBS/12  "AEBSve_d_AEBSwitchStatus_convert"
  Bus_JABS/1 -> JABS_Direct/1(Input_JABS)  "Input_JABS"
  Bus_ELKS/1 -> ELKS_Direct/1(Input_ELKS)  "Input_ELKS"
  LKASve_y_Vehicle_Lane_Display/1 -> Data Type Conversion118/1, ob_In_convert65/1
  Bus_EW/1 -> EW_ISA_TSR_Direct/1(Input_EWWW)  "Input_EWWW"
  JABSve_d_DbFltStatus/1 -> Data Type Conversion173/1, ob_In_convert60/1
  ICABva_d_ICAB2HMI/1 -> Data Type Conversion31/1, ob_In_convert90/1
  Data Type Conversion31/1 -> Bus_ICA/3  "ICABva_d_ICAB2HMI_convert"
  Data Type Conversion80/1 -> Bus_AEBS/25  "AEBSve_d_DAS1_Status_FCW_DBSReq_convert"
  Constant5/1 -> Bus Creator/1  "Input_ESAS"
  Data Type Conversion104/1 -> Bus_IMAP/9  "IMAPve_g_L0_C3_convert"
  Data Type Conversion5/1 -> Bus_AEBS/21  "AEBSve_d_JABS_HapticAlarm_convert"
  Data Type Conversion12/1 -> Bus_ELKS/1  "ELKSve_y_state_ELK_function_convert"
  Data Type Conversion81/1 -> Bus_AEBS/26  "AEBSve_d_DAS3_Status_FCWWarning_Lvl_convert"
  Data Type Conversion94/1 -> Bus_ACCS/2  "ACCSve_g_ACC_TqReq_convert"
  Data Type Conversion106/1 -> Bus_IMAP/11  "IMAPve_g_R0_C1_convert"
  Bus_AEBS/1 -> AEBS_Direct/1(Input_AEBS)  "Input_AEBS"
  Data Type Conversion134/1 -> Bus_EW/15  "EWWWve_y_SRR_SystemState_convert"
  [FD_Input] -> AEBS_Direct/2(Input_FDMM)
  Data Type Conversion131/1 -> Bus_EW/12  "EWWWve_y_SRR_LF_ErrorSt_convert"
  Bus_ICA/1 -> ICA_Direct_G59/1(Input_ICA)  "Input_ICA"
  EWWWve_y_RCTA_M_SystemWorkingSt/1 -> Data Type Conversion121/1, ob_In_convert99/1
  [FD_Input] -> JABS_Direct/2(Input_FDMM)
  Ground9/1 -> ob_In_convert135/1, Data Type Conversion78/1
  Bus_IMAP/1 -> [IMAP_Input]
  Data Type Conversion164/1 -> Bus_JABS/1  "JABSve_d_DbPrefillReq_convert"
  Bus_LKAS/1 -> LKAS_Direct/1(Input_LKAS)  "Input_LKAS"
  [FD_Input] -> ACCS_Direct/2(Input_FDMM)
  [IMAP_Input] -> ACCS_Direct/3(Input_IMAP)
  [FD_Input] -> EW_ISA_TSR_Direct/2(Input_FDMM)
  [FD_Input] -> ICA_Direct_G59/2(Input_FDMM)
  [IMAP_Input] -> ICA_Direct_G59/3(Input_IMAP)
  [ACC_to_ICA] -> ICA_Direct_G59/4(ACC_to_ICA)
  Ground10/1 -> ob_In_convert130/1, Data Type Conversion82/1
  ob_In_convert130/1 -> ob_In_terminator130/1  "ob_OACC_ACC_CtlVeh_LZM"
  ob_In_convert131/1 -> ob_In_terminator131/1  "ob_OACC_ACC_CancelReq_LZM"
  ob_In_convert132/1 -> ob_In_terminator132/1  "ob_OACC_ACC_GoIndicateReq_LZM"
  ob_In_convert133/1 -> ob_In_terminator133/1  "ob_OACC_ACC_OverrideIndReq_LZM"
  ob_In_convert134/1 -> ob_In_terminator134/1  "ob_OACC_ACC_TakeoverIndReq_LZM"
  ob_In_convert135/1 -> ob_In_terminator135/1  "ob_OAEB_DAS1_AEBWarning"
  ob_In_convert136/1 -> ob_In_terminator136/1  "ob_OAEB_DAS1_DBS_Enable"
  ob_In_convert137/1 -> ob_In_terminator137/1  "ob_OAEB_DAS1_FCW_DBSReq"
  ob_In_convert138/1 -> ob_In_terminator138/1  "ob_OAEB_DAS3_FCWWarning"
  ob_In_convert139/1 -> ob_In_terminator139/1  "ob_OLKA_LKATorqueReq"
  ob_In_convert140/1 -> ob_In_terminator140/1  "ob_OLKA_LKATorqueReq_Value"
  ob_In_convert141/1 -> ob_In_terminator141/1  "ob_OELK_LKATorqueReq"
  ob_In_convert142/1 -> ob_In_terminator142/1  "ob_OELK_LKATorqueReq_Value"
  ob_In_convert143/1 -> ob_In_terminator143/1  "ob_OICAB_LKATorqueReq"
  ob_In_convert144/1 -> ob_In_terminator144/1  "ob_OICAB_LKATorqueReq_Value"
  ob_In_convert1/1 -> ob_In_terminator1/1  "ob_OFD_JaFcnConf"
  ob_In_convert2/1 -> ob_In_terminator2/1  "ob_OFD_AebFcnConf"
  ob_In_convert3/1 -> ob_In_terminator3/1  "ob_OFD_EsaFcnConf"
  ob_In_convert4/1 -> ob_In_terminator4/1  "ob_OFD_ElkFcnConf"
  ob_In_convert5/1 -> ob_In_terminator5/1  "ob_OFD_LkaFcnConf"
  ob_In_convert6/1 -> ob_In_terminator6/1  "ob_OFD_IcaFcnConf"
  ob_In_convert7/1 -> ob_In_terminator7/1  "ob_OFD_AccFcnConf"
  ob_In_convert8/1 -> ob_In_terminator8/1  "ob_OFD_LfFcnConf"
  ob_In_convert9/1 -> ob_In_terminator9/1  "ob_OFD_AlcFcnConf"
  ob_In_convert10/1 -> ob_In_terminator10/1  "ob_OFD_EwFcnConf"
  ob_In_convert11/1 -> ob_In_terminator11/1  "ob_OFD_Adas2Fapa"
  ob_In_convert12/1 -> ob_In_terminator12/1  "ob_OFD_SignalTStamp"
  ob_In_convert13/1 -> ob_In_terminator13/1  "ob_OACC_ACC_State"
  ob_In_convert14/1 -> ob_In_terminator14/1  "ob_OACC_ACC_TqReq"
  ob_In_convert15/1 -> ob_In_terminator15/1  "ob_OACC_ACC_TqFlag"
  ob_In_convert16/1 -> ob_In_terminator16/1  "ob_OACC_ACC_DecReq"
  ob_In_convert17/1 -> ob_In_terminator17/1  "ob_OACC_ACC_DecFlag"
  ob_In_convert18/1 -> ob_In_terminator18/1  "ob_OACC_CIPV_ID"
  ob_In_convert19/1 -> ob_In_terminator19/1  "ob_OACC_ACCActive_Signal"
  ob_In_convert20/1 -> ob_In_terminator20/1  "ob_OACC_ACC_go_request"
  ob_In_convert21/1 -> ob_In_terminator21/1  "ob_OACC_VelocitySet"
  ob_In_convert22/1 -> ob_In_terminator22/1  "ob_OACC_HeadWaySet"
  ob_In_convert23/1 -> ob_In_terminator23/1  "ob_OACC_SignalTStamp"
  ob_In_convert24/1 -> ob_In_terminator24/1  "ob_OACC_ACC_ICA_Flag"
  ob_In_convert25/1 -> ob_In_terminator25/1  "ob_OACC_ACC_ESCDriveOff"
  ob_In_convert26/1 -> ob_In_terminator26/1  "ob_OACC_ACC_ESCHoldReq"
  ob_In_convert27/1 -> ob_In_terminator27/1  "ob_OACC_ACC_EPBReq"
  ob_In_convert28/1 -> ob_In_terminator28/1  "ob_OAEB_Prefill_request"
  ob_In_convert29/1 -> ob_In_terminator29/1  "ob_OAEB_functionFARCState"
  ob_In_convert30/1 -> ob_In_terminator30/1  "ob_OAEB_DecSetpoint"
  ob_In_convert31/1 -> ob_In_terminator31/1  "ob_OAEB_MDDdecRequest"
  ob_In_convert32/1 -> ob_In_terminator32/1  "ob_OAEB_MDDdecType"
  ob_In_convert33/1 -> ob_In_terminator33/1  "ob_OAEB_ESCDriveOff"
  ob_In_convert34/1 -> ob_In_terminator34/1  "ob_OAEB_ESCHoldReq"
  ob_In_convert35/1 -> ob_In_terminator35/1  "ob_OAEB_HapticAlarm"
  ob_In_convert36/1 -> ob_In_terminator36/1  "ob_OAEB_Braking_progress"
  ob_In_convert37/1 -> ob_In_terminator37/1  "ob_OAEB_AEBStatus"
  ob_In_convert38/1 -> ob_In_terminator38/1  "ob_OAEB_FCWStatus"
  ob_In_convert39/1 -> ob_In_terminator39/1  "ob_OAEB_AEBSwitchStatus"
  ob_In_convert40/1 -> ob_In_terminator40/1  "ob_OAEB_AEBFaultStatus"
  ob_In_convert41/1 -> ob_In_terminator41/1  "ob_OAEB_AEBAlertReq"
  ob_In_convert42/1 -> ob_In_terminator42/1  "ob_OAEB_AEBTips"
  ob_In_convert43/1 -> ob_In_terminator43/1  "ob_OAEB_SignalTStamp"
  ob_In_convert44/1 -> ob_In_terminator44/1  "ob_OAEB_JABS_AlertSign"
  ob_In_convert45/1 -> ob_In_terminator45/1  "ob_OAEB_JABS_SwitchStatus"
  ob_In_convert46/1 -> ob_In_terminator46/1  "ob_OAEB_JABS_FltStatus"
  ob_In_convert47/1 -> ob_In_terminator47/1  "ob_OAEB_JABS_AlertReq"
  ob_In_convert48/1 -> ob_In_terminator48/1  "ob_OAEB_JABS_HapticAlarm"
  ob_In_convert49/1 -> ob_In_terminator49/1  "ob_OAEB_JABS_Tips"
  ob_In_convert50/1 -> ob_In_terminator50/1  "ob_OJAB_DbPrefillReq"
  ob_In_convert51/1 -> ob_In_terminator51/1  "ob_OJAB_DbFunFARCSta"
  ob_In_convert52/1 -> ob_In_terminator52/1  "ob_OJAB_DbDecSetpoint"
  ob_In_convert53/1 -> ob_In_terminator53/1  "ob_OJAB_DbMDDdecRequest"
  ob_In_convert54/1 -> ob_In_terminator54/1  "ob_OJAB_DbMDDdecType"
  ob_In_convert55/1 -> ob_In_terminator55/1  "ob_OJAB_DbHapticAlarm"
  ob_In_convert56/1 -> ob_In_terminator56/1  "ob_OJAB_DbBraking_progress"
  ob_In_convert57/1 -> ob_In_terminator57/1  "ob_OJAB_DbSignalTStamp"
  ob_In_convert58/1 -> ob_In_terminator58/1  "ob_OJAB_DbJACWStatus"
  ob_In_convert59/1 -> ob_In_terminator59/1  "ob_OJAB_DbSwitchStatus"
  ob_In_convert60/1 -> ob_In_terminator60/1  "ob_OJAB_DbFltStatus"
  ob_In_convert61/1 -> ob_In_terminator61/1  "ob_OJAB_DbAlertReq"
  ob_In_convert62/1 -> ob_In_terminator62/1  "ob_OJAB_DbTips"
  ob_In_convert63/1 -> ob_In_terminator63/1  "ob_OJAB_DbESCDriveOff"
  ob_In_convert64/1 -> ob_In_terminator64/1  "ob_OJAB_DbESCHoldReq"
  ob_In_convert65/1 -> ob_In_terminator65/1  "ob_OLKA_Vehicle_Lane_Display"
  ob_In_convert66/1 -> ob_In_terminator66/1  "ob_OLKA_LDW_Status_Display"
  ob_In_convert67/1 -> ob_In_terminator67/1  "ob_OLKA_LKA_Status_Display"
  ob_In_convert68/1 -> ob_In_terminator68/1  "ob_OLKA_LDW_Flag"
  ob_In_convert69/1 -> ob_In_terminator69/1  "ob_OLKA_Hands_Off_Warning"
  ob_In_convert70/1 -> ob_In_terminator70/1  "ob_OLKA_LKA_Action_Indication"
  ob_In_convert71/1 -> ob_In_terminator71/1  "ob_OLKA_HMI_Popup_Status"
  ob_In_convert72/1 -> ob_In_terminator72/1  "ob_OLKA_EPS_State_Control"
  ob_In_convert73/1 -> ob_In_terminator73/1  "ob_OLKA_LKA_SWA_Control"
  ob_In_convert74/1 -> ob_In_terminator74/1  "ob_OLKA_EPS_Factor_Control"
  ob_In_convert75/1 -> ob_In_terminator75/1  "ob_OLKA_EPS_LKA_Control"
  ob_In_convert76/1 -> ob_In_terminator76/1  "ob_OELK_state_ELK_function"
  ob_In_convert77/1 -> ob_In_terminator77/1  "ob_OELK_ELK_HapticAlarmReq"
  ob_In_convert78/1 -> ob_In_terminator78/1  "ob_OELK_Hands_Off_Warning"
  ob_In_convert79/1 -> ob_In_terminator79/1  "ob_OELK_ELK_Action_Indication"
  ob_In_convert80/1 -> ob_In_terminator80/1  "ob_OELK_HMI_Popup_Status"
  ob_In_convert81/1 -> ob_In_terminator81/1  "ob_OELK_EPS_State_Control"
  ob_In_convert82/1 -> ob_In_terminator82/1  "ob_OELK_ELK_SWA_Control"
  ob_In_convert83/1 -> ob_In_terminator83/1  "ob_OELK_EPS_Factor_Control"
  ob_In_convert84/1 -> ob_In_terminator84/1  "ob_OELK_EPS_ELK_Control"
  ob_In_convert85/1 -> ob_In_terminator85/1  "ob_OELK_ELK_VehicleLaneDisp"
  ob_In_convert86/1 -> ob_In_terminator86/1  "ob_OELK_ELK_ELKSts"
  ob_In_convert87/1 -> ob_In_terminator87/1  "ob_OELK_SignalTStamp"
  ob_In_convert88/1 -> ob_In_terminator88/1  "ob_OICAB_PathQI"
  ob_In_convert89/1 -> ob_In_terminator89/1  "ob_OICAB_SignalTStamp"
  ob_In_convert90/1 -> ob_In_terminator90/1  "ob_OICAB_ICAB2HMI"
  ob_In_convert91/1 -> ob_In_terminator91/1  "ob_OICAB_SteerAngleCmd"
  ob_In_convert92/1 -> ob_In_terminator92/1  "ob_OICAB_ICAMode"
  ob_In_convert93/1 -> ob_In_terminator93/1  "ob_OICAB_ICAState"
  ob_In_convert94/1 -> ob_In_terminator94/1  "ob_OICAD_DecionState"
  ob_In_convert95/1 -> ob_In_terminator95/1  "ob_OICAD_DecionCMD"
  ob_In_convert96/1 -> ob_In_terminator96/1  "ob_OICAD_LCRecommend"
  ob_In_convert97/1 -> ob_In_terminator97/1  "ob_OICAD_SignalTStamp"
  ob_In_convert98/1 -> ob_In_terminator98/1  "ob_OEW_LCW_M_SystemWorkingSt"
  ob_In_convert99/1 -> ob_In_terminator99/1  "ob_OEW_RCTA_M_SystemWorkingSt"
  ob_In_convert100/1 -> ob_In_terminator100/1  "ob_OEW_DOW_M_SystemWorkingSt"
  ob_In_convert101/1 -> ob_In_terminator101/1  "ob_OEW_BSD_M_ErrorSt"
  ob_In_convert102/1 -> ob_In_terminator102/1  "ob_OEW_BSD_M_LCAWarning"
  ob_In_convert103/1 -> ob_In_terminator103/1  "ob_OEW_BSD_M_DoorOpenWarning"
  ob_In_convert104/1 -> ob_In_terminator104/1  "ob_OEW_BSD_M_RCTAWarning"
  ob_In_convert105/1 -> ob_In_terminator105/1  "ob_OEW_BSD_S_LCAWarning"
  ob_In_convert106/1 -> ob_In_terminator106/1  "ob_OEW_BSD_S_DoorOpenWarning"
  ob_In_convert107/1 -> ob_In_terminator107/1  "ob_OEW_BSD_S_RCTAWarning"
  ob_In_convert108/1 -> ob_In_terminator108/1  "ob_OEW_SRR_LF_FCTAWorkingSt"
  ob_In_convert109/1 -> ob_In_terminator109/1  "ob_OEW_SRR_LF_ErrorSt"
  ob_In_convert110/1 -> ob_In_terminator110/1  "ob_OEW_SRR_LF_FCTAWarning"
  ob_In_convert111/1 -> ob_In_terminator111/1  "ob_OEW_SRR_RF_FCTAWarning"
  ob_In_convert112/1 -> ob_In_terminator112/1  "ob_OEW_SRR_SystemState"
  ob_In_convert113/1 -> ob_In_terminator113/1  "ob_OEW_BSD_S_SystemStateInfo"
  ob_In_convert114/1 -> ob_In_terminator114/1  "ob_OEW_BSD_SystemStateInfo"
  ob_In_convert115/1 -> ob_In_terminator115/1  "ob_OEW_SRR_LF_SystemStateInfo"
  ob_In_convert116/1 -> ob_In_terminator116/1  "ob_OEW_SRR_RF_SystemStateInfo"
  ob_In_convert117/1 -> ob_In_terminator117/1  "ob_OIMAP_EPS_LKA_State"
  ob_In_convert118/1 -> ob_In_terminator118/1  "ob_OIMAP_ESC_LonAcc"
  ob_In_convert119/1 -> ob_In_terminator119/1  "ob_OIMAP_obj_id"
  ob_In_convert120/1 -> ob_In_terminator120/1  "ob_OIMAP_obj_pos_x"
  ob_In_convert121/1 -> ob_In_terminator121/1  "ob_OIMAP_ESC_Veh_Standstill"
  ob_In_convert122/1 -> ob_In_terminator122/1  "ob_OIMAP_L0_C0"
  ob_In_convert123/1 -> ob_In_terminator123/1  "ob_OIMAP_L0_C1"
  ob_In_convert124/1 -> ob_In_terminator124/1  "ob_OIMAP_L0_C2"
  ob_In_convert125/1 -> ob_In_terminator125/1  "ob_OIMAP_L0_C3"
  ob_In_convert126/1 -> ob_In_terminator126/1  "ob_OIMAP_R0_C0"
  ob_In_convert127/1 -> ob_In_terminator127/1  "ob_OIMAP_R0_C1"
  ob_In_convert128/1 -> ob_In_terminator128/1  "ob_OIMAP_R0_C2"
  ob_In_convert129/1 -> ob_In_terminator129/1  "ob_OIMAP_R0_C3"
  [ICA_EPS] -> Index Vector2/10
